simulink library "outp"  (R2021b)
settings: Solver=VariableStepAuto  StartTime=0.0  StopTime=10.0  RelTol=1e-3
undefined symbols (not defined in the file or in its folder): ENUM_PMMMODE_CHARGE, ENUM_PMMMODE_IDLE, ENUM_PMMMODE_INITIALIZE, ENUM_PMMMODE_POWERDOWN, ENUM_PMMMODE_SLEEP, Left, outp, slcm, TRUE
libraries: FVT_lib x645, hcu_lib x4, simulink x1
(part 2 of 7)

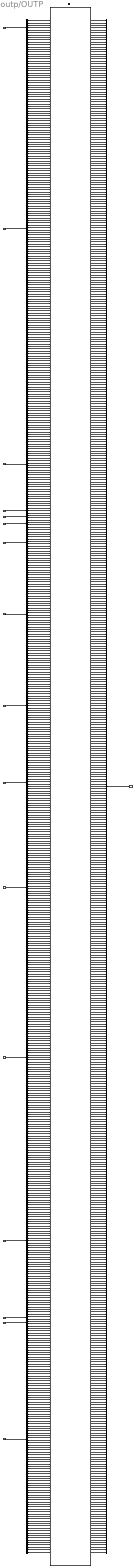
== system outp/OUTP ==
  BACC_outputs : Inport  OutDataTypeStr=Bus: BACC_outputs
  BAPM_outputs : Inport  Port=2  OutDataTypeStr=Bus: BAPM_outputs
  BBCM_outputs : Inport  Port=3  OutDataTypeStr=Bus: BBCM_outputs
  BDHP_outputs : Inport  Port=4  OutDataTypeStr=Bus: BDHP_outputs
  BDKC_outputs : Inport  Port=5  OutDataTypeStr=Bus: BDKC_outputs
  BDSC_outputs : Inport  Port=6  OutDataTypeStr=Bus: BDSC_outputs
  BNMM_outputs : Inport  Port=7  OutDataTypeStr=Bus: BNMM_outputs
  BPMM_outputs : Inport  Port=8  OutDataTypeStr=Bus: BPMM_outputs
  BSCP_outputs : Inport  Port=9  OutDataTypeStr=Bus: BSCP_outputs
  BSYS_outputs : Inport  Port=10  OutDataTypeStr=Bus: BSYS_outputs
  BTHC_outputs : Inport  Port=11  OutDataTypeStr=Bus: BTHC_outputs
  BTPM_outputs : Inport  Port=12  OutDataTypeStr=Bus: BTPM_outputs
  BTQD_outputs : Inport  Port=13  OutDataTypeStr=Bus: BTQD_outputs
  BTQR_outputs : Inport  Port=14  OutDataTypeStr=Bus: BTQR_outputs
  BV2L_outputs : Inport  Port=15  OutDataTypeStr=Bus: BV2L_outputs
  BVMC_outputs : Inport  Port=16  OutDataTypeStr=Bus: BVMC_outputs
  trig_OUTP : TriggerPort  TriggerType=function-call  VariantControl=(inherit)
  bus_creator : BusCreator  Inputs=645
  bus_selector1 : BusSelector  OutputSignals=VACC_HVTHCMSysAvail_enum,VACC_LVBattVoltSta_enum,VACC_VehHVPwrAvail4THCM_W,VACC_EHPSEnDem_enum,VACC_CACPresWarnSta_flg,VACC_CACTempWarnSta_flg,VACC_EACEnDem_enum
  bus_selector10 : BusSelector  OutputSignals=VSYS_HWVer1_cnt,VSYS_HWVer2_cnt,VSYS_HWVer3_cnt,VSYS_CarModel1_cnt,VSYS_CarModel2_cnt,VSYS_CarModel3_cnt,VSYS_ECU1_cnt,VSYS_ECU2_cnt,VSYS_Major1_cnt,VSYS_Major2_cnt,VSYS_Minor1_cnt,VSYS_Minor2_cnt,VSYS_Patch1_cnt,VSYS_Patch2_cnt,VSYS_Country1_cnt,VSYS_Country2_cnt,VSYS_Variation_cnt,VSYS_Dash1_cnt,VSYS_Change1_cnt,VSYS_Change2_cnt,VSYS_Dash2_cnt,VSYS_SHA1_cnt,VSYS_SHA2_cnt,VSYS_SHA3_cnt,VSYS_SHA4_cnt,VSYS_SHA5_cnt,VSYS_SHA6_cnt,VSYS_SHA7_cnt,VSYS_SHA8_cnt,VSYS_NvWriteReqRisingEdge_flg,VSYS_FdcSlpReqRisingEdge_flg,VSYS_FdcSlpTime_sec,VSYS_PmicBootReason_enum,VSYS_WisrBootReason_raw32,VSYS_AcoreRebootCmdACK_flg,VSYS_CurrentNmState_enum
  bus_selector11 : BusSelector  OutputSignals=VTHC_FDCompCmd_rpm,VTHC_FDSOV1Cmd_flg,VTHC_FDSOV2Cmd_flg,VTHC_FDSOV3Cmd_flg,VTHC_FDEXV1Cmd_step,VTHC_FDEXV2Cmd_step,VTHC_FDSOTXVCmd_flg,VTHC_FDFWVCmd_flg,VTHC_FDTWVCmd_pct,VTHC_FDFrWPTCHeatPwrCmd_W,VTHC_CoolgFanActDuty_pct,VTHC_FDAGSCmd_enum,VTHC_FDEWP1Cmd_enum,VTHC_FDEWP2Cmd_enum,VTHC_FDEWP3Cmd_enum,VTHC_FDFrLeAPTCHeatPwrCmd_W,VTHC_FDFrRiAPTCHeatPwrCmd_W,VTHC_FDRrAPTCHeatPwrCmd_W,VTHC_FDBlowerCmd_pct,VTHC_BatteryMode_enum,VTHC_EDriveMode_enum,VTHC_CabinMode_enum,VTHC_CCUACLampSts_flg,VTHC_CCUAutoLampSts_flg,VTHC_CCUACMaxLampSts_flg,VTHC_CCUSyncLampSts_flg,VTHC_sigAirIntenZon1St_enum,VTHC_sigWindDirZon1St_enum,VTHC_sigRecircSt_flg,VTHC_sigSetTempZon1St_C,VTHC_sigSetTempZon2St_C,VTHC_sigClntTHvBattOut_C,VTHC_sigCbnSolarLeft_W,VTHC_sigClntTHvBattIn_C,VTHC_sigCbnSolarRight_W,VTHC_sigAmbAirT_C,VTHC_sigCbnAirT_C,VTHC_ACSubMode_enum,VTHC_FDRecyAutoCmd_enum,VTHC_ACModeMem_enum,VTHC_Face_flg,VTHC_Foot_flg,VTHC_Frost_flg,VTHC_FaceM_flg,VTHC_FootM_flg,VTHC_CCUSyncSts_flg,VTHC_ACForceOFF_flg,VTHC_RecAutoFlg_flg,VTHC_AirIntenZone1M_enum,VTHC_fdefog_flg,VTHC_sigSetTempZon2StM_C,VTHC_FDCTHCMAPTCWarningSta_flg
  bus_selector12 : BusSelector  OutputSignals=VTPM_LFBatWarn_flg,VTPM_RFBatWarn_flg,VTPM_LRBatWarn_flg,VTPM_RRBatWarn_flg,VTPM_LFWheelPress_raw8,VTPM_RFWheelPress_raw8,VTPM_LRWheelPress_raw8,VTPM_RRWheelPress_raw8,VTPM_LFWheelTemp_C,VTPM_RFWheelTemp_C,VTPM_LRWheelTemp_C,VTPM_RRWheelTemp_C,VTPM_LFSensorFail_flg,VTPM_RFSensorFail_flg,VTPM_LRSensorFail_flg,VTPM_RRSensorFail_flg,VTPM_LFWheelDebug_flg,VTPM_LRWheelDebug_flg,VTPM_RFWheelDebug_flg,VTPM_RRWheelDebug_flg,VTPM_TPMSResButtAllow_flg,VTPM_TPMSCaliButtAllow_flg,VTPM_LFPressIndi_enum,VTPM_RFPressIndi_enum,VTPM_LRPressIndi_enum,VTPM_RRPressIndi_enum,VTPM_TPMSWarnIndi_enum,VTPM_LFWheelTmpIndi_flg,VTPM_RFWheelTmpIndi_flg,VTPM_LRWheelTmpIndi_flg,VTPM_RRWheelTmpIndi_flg,VTPM_LFWheelPSW_raw8,VTPM_LRWheelPSW_raw8,VTPM_RFWheelPSW_raw8,VTPM_RRWheelPSW_raw8,VTPM_CWheelTips_enum,VTPM_AutoLTips_enum,VTPM_LFSensorMode_flg,VTPM_RFSensorMode_flg,VTPM_LRSensorMode_flg,VTPM_RRSensorMode_flg,VTPM_S1ID_raw32,VTPM_S2ID_raw32,VTPM_S3ID_raw32,VTPM_S4ID_raw32,VTPM_S1L_enum,VTPM_S2L_enum,VTPM_S3L_enum,VTPM_S4L_enum,VTPM_ALFin_flg,VTPM_LFP20_raw8,VTPM_RFP20_raw8,VTPM_LRP20_raw8,VTPM_RRP20_raw8,VTPM_FAT_flg,VTPM_IDin_raw32,VTPM_S1WheelDebugALTU_pct,VTPM_S2WheelDebugALTU_pct,VTPM_S3WheelDebugALTU_pct,VTPM_S4WheelDebugALTU_pct,VTPM_ID1messageALTU_raw8,VTPM_ID2messageALTU_raw8,VTPM_ID3messageALTU_raw8,VTPM_ID4messageALTU_raw8,VTPM_Chkfin_flg,VTPM_SetIDLoc_flg,VTPM_TPMSStorge_flg,VTPM_ChkStorge_flg,VTPM_TPMSResButt_flg,VTPM_LFPindi_enum,VTPM_RFPind_enum,VTPM_LRPindi_enum,VTPM_RRPindi_enum,VTPM_WriteChkLFID_raw,VTPM_WriteChkRFID_raw,VTPM_WriteChkLRID_raw,VTPM_WriteChkRRID_raw,VTPM_WriteChkfinLFID_raw,VTPM_WriteChkfinRFID_raw,VTPM_WriteChkfinLRID_raw,VTPM_WriteChkfinRRID_raw,VTPM_Flashchkdatavalid_enum,VTPM_Flashdatavalid_enum,VTPM_unlearnSfali_flg,VTPM_unlearnSfailvalid_enum,VTPM_Prepresstempvalid_enum,VTPM_FlashS1ID_raw,VTPM_FlashS2ID_raw,VTPM_FlashS3ID_raw,VTPM_FlashS4ID_raw,VTPM_FlashIDvalid_enum
  bus_selector13 : BusSelector  OutputSignals=VTQD_ParkRequest_flg,VTQD_TqSourceFr_enum,VTQD_TqSourceRr_enum,VTQD_FrEDUAvailBrkRgnTq_Nm,VTQD_RrEDUAvailBrkRgnTq_Nm,VTQD_EVDriveMode_enum,VTQD_ShiftGearPosn_enum,VTQD_PButtonSta_enum,VTQD_FrActvDmpDisabReq_flg,VTQD_RrActvDmpDisabReq_flg,VTQD_FrRgnDecrSta_flg,VTQD_RrRgnDecrSta_flg,VTQD_DriverWhlTqDemFr_Nm,VTQD_DriverWhlTqDemRr_Nm,VTQD_FrEDUActTq_Nm,VTQD_RrEDUActTq_Nm,VTQD_FrEDURolRgnTq_Nm,VTQD_RrEDURolRgnTq_Nm,VTQD_FrEDUSpd_rpm,VTQD_RrEDUSpd_rpm,VTQD_FrEDUSpdValid_flg,VTQD_FrEDUAvailBrkRgnTqV_flg,VTQD_RrEDUSpdValid_flg,VTQD_RrEDUAvailBrkRgnTqV_flg,VTQD_RgnAbnorSta_flg,VTQD_PTCSPermSta_flg,VTQD_FrRgnPermSta_flg,VTQD_RrRgnPermSta_flg,VTQD_FrIdcMin_A,VTQD_FrIdcMax_A,VTQD_FrUdcMin_V,VTQD_FrUdcMax_V,VTQD_RrIdcMin_A,VTQD_RrIdcMax_A,VTQD_RrUdcMin_V,VTQD_RrUdcMax_V,VTQD_ReBrakeLPReq_flg,VTQD_CreepON_flg,VTQD_ActEMpTrq_pct,VTQD_ActMaxAvaEMRecpTrq_pct,VTQD_ActDriveDirect_enum,VTQD_DLEngaged_enum,VTQD_EMTrqModeDrvBrk_enum,VTQD_ActEMpTrqHrls_pct,VTQD_ActEMOutSftSpd_rpm,VTQD_DrvDemEMRtapTrq_pct,VTQD_SACtrlDev_enum,VTQD_RetSelNonEng_pct,VTQD_ShiftPgs_enum,VTQD_AccPedal1LowSW_enum,VTQD_AccPedalPos1_pct,VTQD_ParkBrakeSW_enum,VTQD_VCUVehSpd_kph,VTQD_BrakeSW_enum,VTQD_NFricPercTorq_pct,VTQD_EMParasLoss_pct,VTQD_EEC2MSGCnt_raw,VTQD_EEC2MSGCS_raw,VTQD_FDCCHAEBSRd4BRSta_enum,VTQD_FDCCHAEBSHBSwSta_enum,VTQD_FDCCHAEBSHHSwSta_enum,VTQD_FDCVCUTUpAStaSta_enum,VTQD_FDCVCUDACStatusSta_enum
  bus_selector14 : BusSelector  OutputSignals=VTQR_FrTMTqReq_Nm,VTQR_RrTMTqReq_Nm
  bus_selector15 : BusSelector  OutputSignals=VV2L_ReqOBCV2LEna_enum,VV2L_ReqV2LIVIPopup_enum
  bus_selector16 : BusSelector  OutputSignals=VVMC_FeatSetSpdFinal_raw32,VVMC_VehicleSpeed_mph,VVMC_VehicleSpeed_kph,VVMC_MeterIndSpeed_raw32,VVMC_VMCAEBCtrlAvail_flg,VVMC_VMCACCCtrlAvail_flg,VVMC_VMCCCCtrlAvail_flg,VVMC_VMCMSACtrlAvail_flg,VVMC_FeatArbitrSta_enum,VVMC_FeatReqSpd_kph,VVMC_JerkPCT_pct,VVMC_LimitPCT_pct,VVMC_FrontRearSlipRatioCtrl_flg,VVMC_RearWhlSlipRatioCtrl_flg,VVMC_SingleWhlSlipRatioCtrl_flg,VVMC_LatAccCtrl_flg,VVMC_SafetyCtrl_flg,VVMC_SPD2ACCAct_flg,VVMC_AccCalcuPID_mps2,VVMC_ISOAccLimit_mps2,VVMC_ISODecLimit_mps2,VVMC_ISOJerkLimit_mps3,VVMC_ACCRequiredAccel_mps2,VVMC_DISCReqAcc_mps2,VVMC_FeatArbitrFinal_enum,VVMC_LateralCtrl_flg,VVMC_ADASLKASta_enum,VVMC_LKAStrToqReq_Nm,VVMC_LKATOIFault_flg,VVMC_LKATOIAct_enum,VVMC_ADASAEBReq_enum,VVMC_ADASFaultSta_flg,VVMC_AEBVehHoldReq_flg,VVMC_ACCVehHoldReq_flg,VVMC_ADASDBSReq_enum,VVMC_ADASACCSta_enum,VVMC_ACCObjDist_m,VVMC_ACCObjRelSpd_mps,VVMC_TimeGapLevel_enum,VVMC_ACCJerkUpperLimit_mps3,VVMC_ACCComfortBandUpper_mps2,VVMC_ACCJerkLowerLimit_mps3,VVMC_ACCComfortBandLower_mps2,VVMC_ADASVehSpdLim_raw32,VVMC_ADASShftPosnReqA_flg,VVMC_ADASShftPosnReq_enum,VVMC_ADASForceIdle_flg,VVMC_HazardWarningReq_flg,VVMC_RightTurnLightReq_flg,VVMC_LeftTurnLightReq_flg,VVMC_ADASFCWSta_enum,VVMC_ADASLDWSta_enum,VVMC_ADASFltWrnReq_flg,VVMC_ACCObjDstLvl_enum,VVMC_ForceLowBeam_enum,VVMC_ACCTakeoverReq_flg,VVMC_ADASWarningMsg_enum,VVMC_ADASCAMSpdLim_enum,VVMC_TargetType_enum,VVMC_ADASSLIFSpdLim_enum,VVMC_LKAHODDisplayWarning_flg,VVMC_LKAHODSoundWarning_flg,VVMC_ADASLFCSta_enum,VVMC_ADASLaneModeL_enum,VVMC_ADASLaneModeR_enum,VVMC_ADASSLIFSta_enum,VVMC_ADASISASta_enum,VVMC_ADASLDWMute_flg,VVMC_ADASFCWMute_flg,VVMC_ADASLFCHandsOffWarning_enum,VVMC_LVDADisabled_flg,VVMC_LVDAMuteSta_enum,VVMC_LVDAFailinfo_flg,VVMC_LVDAWarning_flg,VVMC_LVDAACCStatusInformation_flg,VVMC_ADASLFCWarnSound_enum,VVMC_FCMACCmode_enum,VVMC_ADASLanetypeR_enum,VVMC_ADASLanetypeL_enum,VVMC_ADASLanecurveL_raw32,VVMC_ADASLanecurveR_raw32,VVMC_ADASAEBSta_enum,VVMC_FCMLDWRequest_enum,VVMC_FCMLDWFault_flg,VVMC_ACCCtrlAvail_flg,VVMC_ACCPedalOvrd_flg,VVMC_TimeGapCalcu_s,VVMC_CCCtrlSta_enum,VVMC_MSACtrlSta_enum,VVMC_APSCtrlAvail_flg,VVMC_APSStaSys_enum,VVMC_APSDecReqA_flg,VVMC_APSDecReq_mps2,VVMC_APSReq_enum,VVMC_CCMSASpdWar_flg,VVMC_IMUEnaCmd_flg
  bus_selector2 : BusSelector  OutputSignals=VAPM_VehSpeedToAPM_kph,VAPM_VehSpeedTimeOut_flg,VAPM_FSOffSw_enum,VAPM_FSOffSwTimeOut_flg,VAPM_ChrgPlugSta_enum,VAPM_PASDRMR_cm,VAPM_PASDRML_cm,VAPM_PASDRCR_cm,VAPM_PASDRCL_cm,VAPM_PASDFMR_cm,VAPM_PASDFML_cm,VAPM_PASDFCR_cm,VAPM_PASDFCL_cm,VAPM_APSDRLR_cm,VAPM_APSDRLL_cm,VAPM_APSDFLR_cm,VAPM_APSDFLL_cm,VAPM_PASAFCL_enum,VAPM_PASARMR_enum,VAPM_PASARML_enum,VAPM_PASARCR_enum,VAPM_PASARCL_enum,VAPM_PASAFMR_enum,VAPM_PASAFML_enum,VAPM_PASAFCR_enum,VAPM_USSStaRMR_flg,VAPM_USSStaRML_flg,VAPM_USSStaRLR_flg,VAPM_USSStaRLL_flg,VAPM_USSStaRCR_flg,VAPM_USSStaRCL_flg,VAPM_USSStaFMR_flg,VAPM_USSStaFML_flg,VAPM_USSStaFLR_flg,VAPM_USSStaFLL_flg,VAPM_USSStaFCR_flg,VAPM_USSStaFCL_flg,VAPM_Chime_enum,VAPM_SNSRLayout_enum,VAPM_StaFSya_flg,VAPM_ModOperation_enum,VAPM_BrkPedalPosToAPM_pct,VAPM_BrkPedalPosTimeOut_flg,VAPM_LFRawWhlSpeed_kph,VAPM_LFRawWhlSpeedTimeOut_flg,VAPM_RFRawWhlSpeed_kph,VAPM_RFRawWhlSpeedTimeOut_flg,VAPM_LRRawWhlSpeed_kph,VAPM_LRRawWhlSpeedTimeOut_flg,VAPM_RRRawWhlSpeed_kph,VAPM_RRRawWhlSpeedTimeOut_flg,VAPM_LFRawWhlSpeedV_flg,VAPM_LFRawWhlSpeedVTimeOut_flg,VAPM_RFRawWhlSpeedV_flg,VAPM_RFRawWhlSpeedVTimeOut_flg,VAPM_LRRawWhlSpeedV_flg,VAPM_LRRawWhlSpeedVTimeOut_flg,VAPM_RRRawWhlSpeedV_flg,VAPM_RRRawWhlSpeedVTimeOut_flg,VAPM_LFWhlRotDir_enum,VAPM_LFWhlRotDirTimeOut_flg,VAPM_RFWhlRotDir_enum,VAPM_RFWhlRotDirTimeOut_flg,VAPM_LRWhlRotDir_enum,VAPM_LRWhlRotDirTimeOut_flg,VAPM_RRWhlRotDir_enum,VAPM_RRWhlRotDirTimeOut_flg,VAPM_LFPulseCountV_flg,VAPM_LFPulseCountVTimeOut_flg,VAPM_RFPulseCountV_flg,VAPM_RFPulseCountVTimeOut_flg,VAPM_LRPulseCountV_flg,VAPM_LRPulseCountVTimeOut_flg,VAPM_RRPulseCountV_flg,VAPM_RRPulseCountVTimeOut_flg,VAPM_LFPulseCount_enum,VAPM_LFPulseCountTimeOut_flg,VAPM_RFPulseCount_enum,VAPM_RFPulseCountTimeOut_flg,VAPM_LRPulseCount_enum,VAPM_LRPulseCountTimeOut_flg,VAPM_RRPulseCount_enum,VAPM_RRPulseCountTimeOut_flg,VAPM_ShifterHandleCmd_enum,VAPM_ShifterHandleCmdTimeOut_flg,VAPM_DriIntend_enum,VAPM_DriIntendTimeOut_flg,VAPM_EPSAOIControl_enum,VAPM_EPSAOIControlTimeOut_flg,VAPM_SASAngle_Deg,VAPM_SASAngleTimeOut_flg,VAPM_SASSpeed_degps,VAPM_SASSpeedTimeOut_flg,VAPM_SASSpeedValid_flg,VAPM_SASSpeedValidTimeOut_flg,VAPM_SASCAL_flg,VAPM_SASCALTimeOut_flg,VAPM_SASV_flg,VAPM_SASVTimeOut_flg,VAPM_GRADE_Deg,VAPM_GRADETimeOut_flg,VAPM_YawRate_degps,VAPM_YawRateTimeOut_flg,VAPM_LatAccel_Gps,VAPM_LatAccelTimeOut_flg,VAPM_LongAccel_Gps,VAPM_LongAccelTimeOut_flg,VAPM_MCPressure_bar,VAPM_MCPressureTimeOut_flg,VAPM_YawRateV_flg,VAPM_YawRateVTimeOut_flg,VAPM_LatAccelV_flg,VAPM_LatAccelVTimeOut_flg,VAPM_LongAccelV_flg,VAPM_LongAccelVTimeOut_flg,VAPM_MCPressureV_bar,VAPM_MCPressureVTimeOut_flg,VAPM_BrkSwSta_flg,VAPM_BrkSwStaTimeOut_flg,VAPM_BrkSwV_flg,VAPM_BrkSwVTimeOut_flg,VAPM_ESCStandstill_flg,VAPM_ESCStandstillTimeOut_flg,VAPM_ESCAPSSta_enum,VAPM_ESCAPSStaTimeOut_flg,VAPM_EPBExtReleaseAvail_flg,VAPM_EPBExtReleaseAvailTimeOut_flg,VAPM_EPBExtApplyAvail_flg,VAPM_EPBExtApplyAvailTimeOut_flg,VAPM_EPBErrSta_enum,VAPM_EPBErrStaTimeOut_flg,VAPM_EPBSta_enum,VAPM_EPBStaTimeOut_flg,VAPM_AVMparkingcancel_enum,VAPM_AVMparkingcancelTimeOut_flg,VAPM_AVMparkingexcute_enum,VAPM_AVMparkingexcuteTimeOut_flg,VAPM_AVMParkingmode_enum,VAPM_AVMParkingmodeTimeOut_flg,VAPM_AVMErrSTA_flg,VAPM_AVMErrSTATimeOut_flg,VAPM_IVIStatus_flg,VAPM_IVIStatusTimeOut_flg,VAPM_CAASSw_enum,VAPM_CAASSwTimeOut_flg,VAPM_IVIScreen_enum,VAPM_IVIScreenTimeOut_flg,VAPM_ABSActiveToAPM_flg,VAPM_ABSActiveTimeOut_flg,VAPM_TCSActiveToAPM_flg,VAPM_TCSActiveTimeOut_flg,VAPM_DriverSeatBeltCmd_flg,VAPM_DriverSeatBeltCmdTimeOut_flg,VAPM_APSProgressPCT_pct,VAPM_APSRQDisplay_enum,VAPM_APSSWVer_enum,VAPM_APSHWVer_enum,VAPM_APSExitCondition_enum,VAPM_APSAngleTarget_Deg,VAPM_APSVRqEPASCtrl_flg,VAPM_APSRqEPASCtrl_flg,VAPM_CAASSta_enum
  bus_selector3 : BusSelector  OutputSignals=VBCM_HornCtrl_flg,VBCM_FRHaltBrakeSta_enum,VBCM_FRDisIntEmCmd_flg,VBCM_FROpenClosePBCmd_enum,VBCM_DoorStaSta_enum,VBCM_BrakeLamp_flg,VBCM_LDRL_flg,VBCM_RDRL_flg,VBCM_ReverseLamp_flg,VBCM_RrFogLamp_flg,VBCM_HBeam_flg,VBCM_LBeam_flg,VBCM_PosLamp_flg,VBCM_HazardSW_flg,VBCM_LTurnLP_flg,VBCM_RTurnLP_flg,VBCM_LSMLPCmd_flg,VBCM_RSMLPCmd_flg,VBCM_TurnLpLActiveCmd_flg,VBCM_TurnLpRActiveCmd_flg,VBCM_BBuzzerCmd_flg,VBCM_FrWiperL_flg,VBCM_FrWiperH_flg,VBCM_WasherCtrl_enum,VBCM_RrRmLampBrightCmd_enum,VBCM_WelcomeDemoSta_flg,VBCM_FrAtmoLampCmd_flg,VBCM_RrAtmoLampCmd_flg,VBCM_TgateHDSWLSta_flg,VBCM_TgateHDSWRSta_flg,VBCM_TgateSWLSta_flg,VBCM_TgateSWRSta_flg,VBCM_LTgateRelCmd_flg,VBCM_RTgateRelCmd_flg,VBCM_FDDoorOpen_enum,VBCM_FDDoorstate_enum
  bus_selector4 : BusSelector  OutputSignals=VDHP_ActAPSPosn_pct,VDHP_EAPS1MIN_pct,VDHP_EAPS2MIN_pct
  bus_selector5 : BusSelector  OutputSignals=VDKC_DKCTimeSN_cnt,VDKC_DKCAuthSta_enum
  bus_selector6 : BusSelector  OutputSignals=VDSC_DISCTurn_flg,VDSC_DISCTargetSpd_kph,VDSC_DISCSta_enum,VDSC_DISCButtSta_flg
  bus_selector7 : BusSelector  OutputSignals=VNMM_AllCANTxReq_flg,VNMM_NMmTxReq_flg,VNMM_Awake_enum,VNMM_CSB_flg,VNMM_ErrorState_enum,VNMM_NodeID_enum,VNMM_PNI_flg,VNMM_RptMsgReq_flg,VNMM_WakeUp_enum,VNMM_ActiveWU_flg,VNMM_SysNMmSta_enum,VNMM_NetworkReq_flg
  bus_selector8 : BusSelector  OutputSignals=VPMM_PowerUpState_enum,VPMM_PowerDownState_enum,VPMM_PowerUpFault_enum,VPMM_PowerDownFault_enum,VPMM_ActiveDischargeReq_flg,VPMM_DCDCEnaReq_flg,VPMM_DCDCVoltSetpoint_V,VPMM_HVBatCnctReq_flg,VPMM_HVSysReadyToCharge_enum,VPMM_PowerSta_enum,VPMM_LVPwrSta_flg,VPMM_HVPwrSta_flg,VPMM_SysPowerMode_enum,VPMM_FrMCUEnaReq_flg,VPMM_RrMCUEnaReq_flg,VPMM_DrivetrainSelect_enum,VPMM_DrSeatSta_enum,VPMM_PwrStaSelect_enum,VPMM_PwrStaConstraint_enum,VPMM_TCountSta_enum,VPMM_PwrUpReq_enum,VPMM_PwrDownReq_enum,VPMM_LowSOCWarn_enum,VPMM_ReVehThdChkSta_enum,VPMM_LVSysErrPwrOutErr_flg,VPMM_EvccAplusPwrUpReq_flg,VPMM_PwrStaONTOPopReq_flg,VPMM_IVIPwrStaONTOPopT_s,VPMM_LVChrgHoldTtimer_s,VPMM_LVBattChrgTimeCnt_s,VPMM_SilentChkAllowSleep_flg,VPMM_TimerAllowSleep_flg,VPMM_FDADC12VDetAvg_mV,VPMM_PMMAllowECUSleep_flg,VPMM_LVSilentChrgSta_enum,VPMM_LVSilentChrgReq_flg,VPMM_LVSilentChrgLv_enum,VPMM_CtrlFrPwrStbA1P_flg,VPMM_CtrlFrRC1_flg,VPMM_CtrlFrBMSCCUCIR_flg,VPMM_CtrlFrEDUINVERTER_flg,VPMM_HWResetSta_enum,VPMM_CtrlDrPwrStbA2_flg,VPMM_PwrStaTOSta_enum,VPMM_DCDCRlyDem_enum,VPMM_EACRlyDem_enum,VPMM_EHPSRlyDem_enum,VPMM_DCDCEnDem_enum
  bus_selector9 : BusSelector  OutputSignals=VSCP_Vehspeed_kph,VSCP_SCPBrkSwSta_flg,VSCP_AmberWnlmpSta_flg,VSCP_ABSWnlmpSta_flg,VSCP_HSAFailed_flg,VSCP_MeterIndVehSpeed_kph,VSCP_ABSFailed_flg,VSCP_ABSActive_flg,VSCP_HSAActive_flg,VSCP_RedWnlmpSta_flg,VSCP_BrkPedalPos_pct,VSCP_OpenStatusOfDoor1_enum,VSCP_OpenStatusOfDoor2_enum,VSCP_SeatBeltSwitch_enum,VSCP_triggerBAM_flg,VSCP_CFGEM1Ctrl_raw,VSCP_CFGEM1BAMTSize_raw,VSCP_CFGEM1BAMTNum_raw,VSCP_CFGEM1BAMRsv_raw,VSCP_CFGEM1BAMPGN_raw,VSCP_triggerDT_flg,VSCP_DTbyte0_raw,VSCP_DTbyte1_raw,VSCP_DTbyte2_raw,VSCP_DTbyte3_raw,VSCP_DTbyte4_raw,VSCP_DTbyte5_raw,VSCP_DTbyte6_raw,VSCP_DTbyte7_raw
  outpmodule : Subsystem
  BOUTP_outputs : Outport  OutDataTypeStr=Bus: BOUTP_outputs
  wires:
  outpmodule/33(VOUTP_USSStaRMR_flg) -> bus_creator/33
  outpmodule/32(VOUTP_PASAFCR_enum) -> bus_creator/32
  outpmodule/30(VOUTP_PASAFMR_enum) -> bus_creator/30
  outpmodule/31(VOUTP_PASAFML_enum) -> bus_creator/31
  outpmodule/29(VOUTP_PASARCL_enum) -> bus_creator/29
  outpmodule/28(VOUTP_PASARCR_enum) -> bus_creator/28
  outpmodule/25(VOUTP_PASAFCL_enum) -> bus_creator/25
  outpmodule/23(VOUTP_APSDFLR_cm) -> bus_creator/23
  outpmodule/22(VOUTP_APSDRLL_cm) -> bus_creator/22
  outpmodule/24(VOUTP_APSDFLL_cm) -> bus_creator/24
  outpmodule/21(VOUTP_APSDRLR_cm) -> bus_creator/21
  outpmodule/18(VOUTP_PASDFML_cm) -> bus_creator/18
  outpmodule/16(VOUTP_PASDRCL_cm) -> bus_creator/16
  outpmodule/13(VOUTP_PASDRMR_cm) -> bus_creator/13
  outpmodule/10(VOUTP_FSOffSw_enum) -> bus_creator/10
  outpmodule/9(VOUTP_VehSpeedTimeOut_flg) -> bus_creator/9
  outpmodule/7(VOUTP_EACEnDem_enum) -> bus_creator/7
  outpmodule/6(VOUTP_CACTempWarnSta_flg) -> bus_creator/6
  outpmodule/5(VOUTP_CACPresWarnSta_flg) -> bus_creator/5
  outpmodule/4(VOUTP_EHPSEnDem_enum) -> bus_creator/4
  outpmodule/3(VOUTP_VehHVPwrAvail4THCM_W) -> bus_creator/3
  outpmodule/1(VOUTP_HVTHCMSysAvail_enum) -> bus_creator/1
  outpmodule/378(VOUTP_FDRecyAutoCmd_enum) -> bus_creator/378
  outpmodule/377(VOUTP_ACSubMode_enum) -> bus_creator/377
  outpmodule/374(VOUTP_sigCbnSolarRight_W) -> bus_creator/374
  outpmodule/376(VOUTP_sigCbnAirT_C) -> bus_creator/376
  outpmodule/372(VOUTP_sigCbnSolarLeft_W) -> bus_creator/372
  outpmodule/371(VOUTP_sigClntTHvBattOut_C) -> bus_creator/371
  outpmodule/369(VOUTP_sigSetTempZon1St_C) -> bus_creator/369
  outpmodule/368(VOUTP_sigRecircSt_flg) -> bus_creator/368
  outpmodule/367(VOUTP_sigWindDirZon1St_enum) -> bus_creator/367
  outpmodule/365(VOUTP_CCUSyncLampSts_flg) -> bus_creator/365
  outpmodule/364(VOUTP_CCUACMaxLampSts_flg) -> bus_creator/364
  outpmodule/361(VOUTP_CabinMode_enum) -> bus_creator/361
  outpmodule/359(VOUTP_BatteryMode_enum) -> bus_creator/359
  outpmodule/360(VOUTP_EDriveMode_enum) -> bus_creator/360
  outpmodule/357(VOUTP_FDRrAPTCHeatPwrCmd_W) -> bus_creator/357
  outpmodule/354(VOUTP_FDEWP3Cmd_enum) -> bus_creator/354
  outpmodule/355(VOUTP_FDFrLeAPTCHeatPwrCmd_W) -> bus_creator/355
  outpmodule/353(VOUTP_FDEWP2Cmd_enum) -> bus_creator/353
  outpmodule/350(VOUTP_CoolgFanActDuty_pct) -> bus_creator/350
  outpmodule/347(VOUTP_FDFWVCmd_flg) -> bus_creator/347
  outpmodule/346(VOUTP_FDSOTXVCmd_flg) -> bus_creator/346
  outpmodule/345(VOUTP_FDEXV2Cmd_step) -> bus_creator/345
  outpmodule/344(VOUTP_FDEXV1Cmd_step) -> bus_creator/344
  outpmodule/343(VOUTP_FDSOV3Cmd_flg) -> bus_creator/343
  outpmodule/600(VOUTP_ADASFCWSta_enum) -> bus_creator/600
  outpmodule/381(VOUTP_Foot_flg) -> bus_creator/381
  bus_selector2/43 -> outpmodule/50(VAPM_BrkPedalPosTimeOut_flg)  "<VAPM_BrkPedalPosTimeOut_flg>"
  bus_selector2/46 -> outpmodule/53(VAPM_RFRawWhlSpeed_kph)  "<VAPM_RFRawWhlSpeed_kph>"
  bus_selector2/41 -> outpmodule/48(VAPM_ModOperation_enum)  "<VAPM_ModOperation_enum>"
  bus_selector2/40 -> outpmodule/47(VAPM_StaFSya_flg)  "<VAPM_StaFSya_flg>"
  bus_selector2/136 -> outpmodule/143(VAPM_AVMparkingexcute_enum)  "<VAPM_AVMparkingexcute_enum>"
  bus_selector2/49 -> outpmodule/56(VAPM_LRRawWhlSpeedTimeOut_flg)  "<VAPM_LRRawWhlSpeedTimeOut_flg>"
  bus_selector2/103 -> outpmodule/110(VAPM_YawRateTimeOut_flg)  "<VAPM_YawRateTimeOut_flg>"
  bus_selector2/47 -> outpmodule/54(VAPM_RFRawWhlSpeedTimeOut_flg)  "<VAPM_RFRawWhlSpeedTimeOut_flg>"
  outpmodule/373(VOUTP_sigClntTHvBattIn_C) -> bus_creator/373
  outpmodule/34(VOUTP_USSStaRML_flg) -> bus_creator/34
  bus_selector2/48 -> outpmodule/55(VAPM_LRRawWhlSpeed_kph)  "<VAPM_LRRawWhlSpeed_kph>"
  bus_selector2/45 -> outpmodule/52(VAPM_LFRawWhlSpeedTimeOut_flg)  "<VAPM_LFRawWhlSpeedTimeOut_flg>"
  outpmodule/184(VOUTP_LTurnLP_flg) -> bus_creator/184
  outpmodule/185(VOUTP_RTurnLP_flg) -> bus_creator/185
  outpmodule/183(VOUTP_HazardSW_flg) -> bus_creator/183
  outpmodule/182(VOUTP_PosLamp_flg) -> bus_creator/182
  outpmodule/178(VOUTP_ReverseLamp_flg) -> bus_creator/178
  bus_selector2/35 -> outpmodule/42(VAPM_USSStaFLL_flg)  "<VAPM_USSStaFLL_flg>"
  outpmodule/176(VOUTP_LDRL_flg) -> bus_creator/176
  outpmodule/174(VOUTP_DoorStaSta_enum) -> bus_creator/174
  outpmodule/173(VOUTP_FROpenClosePBCmd_enum) -> bus_creator/173
  outpmodule/172(VOUTP_FRDisIntEmCmd_flg) -> bus_creator/172
  outpmodule/170(VOUTP_HornCtrl_flg) -> bus_creator/170
  outpmodule/169(VOUTP_CAASSta_enum) -> bus_creator/169
  outpmodule/168(VOUTP_APSRqEPASCtrl_flg) -> bus_creator/168
  outpmodule/237(VOUTP_LVPwrSta_flg) -> bus_creator/237
  outpmodule/175(VOUTP_BrakeLamp_flg) -> bus_creator/175
  outpmodule/234(VOUTP_HVBatCnctReq_flg) -> bus_creator/234
  outpmodule/236(VOUTP_PowerSta_enum) -> bus_creator/236
  outpmodule/232(VOUTP_DCDCEnaReq_flg) -> bus_creator/232
  outpmodule/228(VOUTP_PowerDownState_enum) -> bus_creator/228
  outpmodule/225(VOUTP_SysNMmSta_enum) -> bus_creator/225
  outpmodule/224(VOUTP_ActiveWU_flg) -> bus_creator/224
  outpmodule/222(VOUTP_RptMsgReq_flg) -> bus_creator/222
  outpmodule/220(VOUTP_NodeID_enum) -> bus_creator/220
  outpmodule/218(VOUTP_CSB_flg) -> bus_creator/218
  outpmodule/217(VOUTP_Awake_enum) -> bus_creator/217
  outpmodule/216(VOUTP_NMmTxReq_flg) -> bus_creator/216
  outpmodule/215(VOUTP_AllCANTxReq_flg) -> bus_creator/215
  outpmodule/214(VOUTP_DISCButtSta_flg) -> bus_creator/214
  outpmodule/212(VOUTP_DISCTargetSpd_kph) -> bus_creator/212
  outpmodule/210(VOUTP_DKCAuthSta_enum) -> bus_creator/210
  outpmodule/207(VOUTP_EAPS1MIN_pct) -> bus_creator/207
  outpmodule/206(VOUTP_ActAPSPosn_pct) -> bus_creator/206
  outpmodule/205(VOUTP_FDDoorstate_enum) -> bus_creator/205
  outpmodule/204(VOUTP_FDDoorOpen_enum) -> bus_creator/204
  outpmodule/198(VOUTP_TgateHDSWLSta_flg) -> bus_creator/198
  outpmodule/196(VOUTP_FrAtmoLampCmd_flg) -> bus_creator/196
  outpmodule/195(VOUTP_WelcomeDemoSta_flg) -> bus_creator/195
  outpmodule/193(VOUTP_WasherCtrl_enum) -> bus_creator/193
  outpmodule/192(VOUTP_FrWiperH_flg) -> bus_creator/192
  outpmodule/190(VOUTP_BBuzzerCmd_flg) -> bus_creator/190
  outpmodule/187(VOUTP_RSMLPCmd_flg) -> bus_creator/187
  outpmodule/188(VOUTP_TurnLpLActiveCmd_flg) -> bus_creator/188
  outpmodule/272(VOUTP_EACRlyDem_enum) -> bus_creator/272
  outpmodule/270(VOUTP_PwrStaTOSta_enum) -> bus_creator/270
  outpmodule/269(VOUTP_CtrlDrPwrStbA2_flg) -> bus_creator/269
  outpmodule/267(VOUTP_CtrlFrEDUINVERTER_flg) -> bus_creator/267
  outpmodule/265(VOUTP_CtrlFrRC1_flg) -> bus_creator/265
  outpmodule/264(VOUTP_CtrlFrPwrStbA1P_flg) -> bus_creator/264
  outpmodule/262(VOUTP_LVSilentChrgReq_flg) -> bus_creator/262
  outpmodule/261(VOUTP_LVSilentChrgSta_enum) -> bus_creator/261
  outpmodule/258(VOUTP_TimerAllowSleep_flg) -> bus_creator/258
  outpmodule/259(VOUTP_FDADC12VDetAvg_mV) -> bus_creator/259
  outpmodule/257(VOUTP_SilentChkAllowSleep_flg) -> bus_creator/257
  outpmodule/256(VOUTP_LVBattChrgTimeCnt_s) -> bus_creator/256
  outpmodule/250(VOUTP_ReVehThdChkSta_enum) -> bus_creator/250
  outpmodule/249(VOUTP_LowSOCWarn_enum) -> bus_creator/249
  outpmodule/246(VOUTP_TCountSta_enum) -> bus_creator/246
  outpmodule/244(VOUTP_PwrStaSelect_enum) -> bus_creator/244
  outpmodule/245(VOUTP_PwrStaConstraint_enum) -> bus_creator/245
  outpmodule/241(VOUTP_RrMCUEnaReq_flg) -> bus_creator/241
  outpmodule/300(VOUTP_DTbyte4_raw) -> bus_creator/300
  outpmodule/294(VOUTP_CFGEM1BAMPGN_raw) -> bus_creator/294
  outpmodule/290(VOUTP_CFGEM1Ctrl_raw) -> bus_creator/290
  outpmodule/289(VOUTP_triggerBAM_flg) -> bus_creator/289
  outpmodule/288(VOUTP_SeatBeltSwitch_enum) -> bus_creator/288
  outpmodule/287(VOUTP_OpenStatusOfDoor2_enum) -> bus_creator/287
  outpmodule/285(VOUTP_BrkPedalPos_pct) -> bus_creator/285
  outpmodule/286(VOUTP_OpenStatusOfDoor1_enum) -> bus_creator/286
  outpmodule/278(VOUTP_ABSWnlmpSta_flg) -> bus_creator/278
  outpmodule/275(VOUTP_Vehspeed_kph) -> bus_creator/275
  outpmodule/274(VOUTP_DCDCEnDem_enum) -> bus_creator/274
  bus_selector10/30 -> outpmodule/333(VSYS_NvWriteReqRisingEdge_flg)  "<VSYS_NvWriteReqRisingEdge_flg>"
  bus_selector10/26 -> outpmodule/329(VSYS_SHA5_cnt)  "<VSYS_SHA5_cnt>"
  bus_selector10/25 -> outpmodule/328(VSYS_SHA4_cnt)  "<VSYS_SHA4_cnt>"
  bus_selector10/22 -> outpmodule/325(VSYS_SHA1_cnt)  "<VSYS_SHA1_cnt>"
  bus_selector10/23 -> outpmodule/326(VSYS_SHA2_cnt)  "<VSYS_SHA2_cnt>"
  bus_selector10/20 -> outpmodule/323(VSYS_Change2_cnt)  "<VSYS_Change2_cnt>"
  bus_selector10/18 -> outpmodule/321(VSYS_Dash1_cnt)  "<VSYS_Dash1_cnt>"
  bus_selector10/19 -> outpmodule/322(VSYS_Change1_cnt)  "<VSYS_Change1_cnt>"
  bus_selector10/13 -> outpmodule/316(VSYS_Patch1_cnt)  "<VSYS_Patch1_cnt>"
  outpmodule/252(VOUTP_EvccAplusPwrUpReq_flg) -> bus_creator/252
  bus_selector10/15 -> outpmodule/318(VSYS_Country1_cnt)  "<VSYS_Country1_cnt>"
  bus_selector10/16 -> outpmodule/319(VSYS_Country2_cnt)  "<VSYS_Country2_cnt>"
  bus_selector10/14 -> outpmodule/317(VSYS_Patch2_cnt)  "<VSYS_Patch2_cnt>"
  outpmodule/160(VOUTP_DriverSeatBeltCmdTimeOut_flg) -> bus_creator/160
  outpmodule/167(VOUTP_APSVRqEPASCtrl_flg) -> bus_creator/167
  outpmodule/164(VOUTP_APSHWVer_enum) -> bus_creator/164
  outpmodule/166(VOUTP_APSAngleTarget_Deg) -> bus_creator/166
  outpmodule/165(VOUTP_APSExitCondition_enum) -> bus_creator/165
  outpmodule/340(VOUTP_FDCompCmd_rpm) -> bus_creator/340
  outpmodule/337(VOUTP_WisrBootReason_raw32) -> bus_creator/337
  outpmodule/336(VOUTP_PmicBootReason_enum) -> bus_creator/336
  outpmodule/292(VOUTP_CFGEM1BAMTNum_raw) -> bus_creator/292
  outpmodule/333(VOUTP_NvWriteReqRisingEdge_flg) -> bus_creator/333
  outpmodule/331(VOUTP_SHA7_cnt) -> bus_creator/331
  outpmodule/213(VOUTP_DISCSta_enum) -> bus_creator/213
  outpmodule/332(VOUTP_SHA8_cnt) -> bus_creator/332
  outpmodule/342(VOUTP_FDSOV2Cmd_flg) -> bus_creator/342
  outpmodule/329(VOUTP_SHA5_cnt) -> bus_creator/329
  outpmodule/327(VOUTP_SHA3_cnt) -> bus_creator/327
  outpmodule/326(VOUTP_SHA2_cnt) -> bus_creator/326
  outpmodule/276(VOUTP_SCPBrkSwSta_flg) -> bus_creator/276
  outpmodule/324(VOUTP_Dash2_cnt) -> bus_creator/324
  outpmodule/323(VOUTP_Change2_cnt) -> bus_creator/323
  outpmodule/320(VOUTP_Variation_cnt) -> bus_creator/320
  outpmodule/319(VOUTP_Country2_cnt) -> bus_creator/319
  outpmodule/318(VOUTP_Country1_cnt) -> bus_creator/318
  outpmodule/313(VOUTP_Major2_cnt) -> bus_creator/313
  outpmodule/311(VOUTP_ECU2_cnt) -> bus_creator/311
  outpmodule/309(VOUTP_CarModel3_cnt) -> bus_creator/309
  outpmodule/310(VOUTP_ECU1_cnt) -> bus_creator/310
  bus_selector16/22 -> outpmodule/571(VVMC_ISOJerkLimit_mps3)  "<VVMC_ISOJerkLimit_mps3>"
  bus_selector16/21 -> outpmodule/570(VVMC_ISODecLimit_mps2)  "<VVMC_ISODecLimit_mps2>"
  bus_selector16/20 -> outpmodule/569(VVMC_ISOAccLimit_mps2)  "<VVMC_ISOAccLimit_mps2>"
  bus_selector16/90 -> outpmodule/639(VVMC_APSCtrlAvail_flg)  "<VVMC_APSCtrlAvail_flg>"
  bus_selector16/91 -> outpmodule/640(VVMC_APSStaSys_enum)  "<VVMC_APSStaSys_enum>"
  bus_selector16/92 -> outpmodule/641(VVMC_APSDecReqA_flg)  "<VVMC_APSDecReqA_flg>"
  bus_selector10/29 -> outpmodule/332(VSYS_SHA8_cnt)  "<VSYS_SHA8_cnt>"
  bus_selector16/88 -> outpmodule/637(VVMC_CCCtrlSta_enum)  "<VVMC_CCCtrlSta_enum>"
  bus_selector16/87 -> outpmodule/636(VVMC_TimeGapCalcu_s)  "<VVMC_TimeGapCalcu_s>"
  bus_selector16/84 -> outpmodule/633(VVMC_FCMLDWFault_flg)  "<VVMC_FCMLDWFault_flg>"
  bus_selector16/80 -> outpmodule/629(VVMC_ADASLanecurveL_raw32)  "<VVMC_ADASLanecurveL_raw32>"
  bus_selector16/76 -> outpmodule/625(VVMC_ADASLFCWarnSound_enum)  "<VVMC_ADASLFCWarnSound_enum>"
  bus_selector16/74 -> outpmodule/623(VVMC_LVDAWarning_flg)  "<VVMC_LVDAWarning_flg>"
  bus_selector16/71 -> outpmodule/620(VVMC_LVDADisabled_flg)  "<VVMC_LVDADisabled_flg>"
  bus_selector16/69 -> outpmodule/618(VVMC_ADASFCWMute_flg)  "<VVMC_ADASFCWMute_flg>"
  bus_selector16/65 -> outpmodule/614(VVMC_ADASLaneModeR_enum)  "<VVMC_ADASLaneModeR_enum>"
  bus_selector16/59 -> outpmodule/608(VVMC_TargetType_enum)  "<VVMC_TargetType_enum>"
  bus_selector16/56 -> outpmodule/605(VVMC_ACCTakeoverReq_flg)  "<VVMC_ACCTakeoverReq_flg>"
  bus_selector16/47 -> outpmodule/596(VVMC_ADASForceIdle_flg)  "<VVMC_ADASForceIdle_flg>"
  bus_selector16/49 -> outpmodule/598(VVMC_RightTurnLightReq_flg)  "<VVMC_RightTurnLightReq_flg>"
  bus_selector16/50 -> outpmodule/599(VVMC_LeftTurnLightReq_flg)  "<VVMC_LeftTurnLightReq_flg>"
  bus_selector16/48 -> outpmodule/597(VVMC_HazardWarningReq_flg)  "<VVMC_HazardWarningReq_flg>"
  bus_selector16/42 -> outpmodule/591(VVMC_ACCJerkLowerLimit_mps3)  "<VVMC_ACCJerkLowerLimit_mps3>"
  bus_selector16/44 -> outpmodule/593(VVMC_ADASVehSpdLim_raw32)  "<VVMC_ADASVehSpdLim_raw32>"
  bus_selector16/40 -> outpmodule/589(VVMC_ACCJerkUpperLimit_mps3)  "<VVMC_ACCJerkUpperLimit_mps3>"
  bus_selector16/37 -> outpmodule/586(VVMC_ACCObjDist_m)  "<VVMC_ACCObjDist_m>"
  bus_selector16/38 -> outpmodule/587(VVMC_ACCObjRelSpd_mps)  "<VVMC_ACCObjRelSpd_mps>"
  bus_selector16/34 -> outpmodule/583(VVMC_ACCVehHoldReq_flg)  "<VVMC_ACCVehHoldReq_flg>"
  bus_selector16/32 -> outpmodule/581(VVMC_ADASFaultSta_flg)  "<VVMC_ADASFaultSta_flg>"
  outpmodule/312(VOUTP_Major1_cnt) -> bus_creator/312
  bus_selector16/28 -> outpmodule/577(VVMC_LKAStrToqReq_Nm)  "<VVMC_LKAStrToqReq_Nm>"
  bus_selector10/21 -> outpmodule/324(VSYS_Dash2_cnt)  "<VSYS_Dash2_cnt>"
  bus_selector16/27 -> outpmodule/576(VVMC_ADASLKASta_enum)  "<VVMC_ADASLKASta_enum>"
  bus_selector16/25 -> outpmodule/574(VVMC_FeatArbitrFinal_enum)  "<VVMC_FeatArbitrFinal_enum>"
  bus_selector16/26 -> outpmodule/575(VVMC_LateralCtrl_flg)  "<VVMC_LateralCtrl_flg>"
  bus_selector2/39 -> outpmodule/46(VAPM_SNSRLayout_enum)  "<VAPM_SNSRLayout_enum>"
  outpmodule/200(VOUTP_TgateSWLSta_flg) -> bus_creator/200
  outpmodule/399(VOUTP_RRWheelPress_raw8) -> bus_creator/399
  outpmodule/394(VOUTP_LRBatWarn_flg) -> bus_creator/394
  outpmodule/392(VOUTP_LFBatWarn_flg) -> bus_creator/392
  outpmodule/391(VOUTP_FDCTHCMAPTCWarningSta_flg) -> bus_creator/391
  outpmodule/388(VOUTP_AirIntenZone1M_enum) -> bus_creator/388
  outpmodule/386(VOUTP_ACForceOFF_flg) -> bus_creator/386
  outpmodule/385(VOUTP_CCUSyncSts_flg) -> bus_creator/385
  outpmodule/384(VOUTP_FootM_flg) -> bus_creator/384
  outpmodule/383(VOUTP_FaceM_flg) -> bus_creator/383
  outpmodule/449(VOUTP_S2WheelDebugALTU_pct) -> bus_creator/449
  outpmodule/448(VOUTP_S1WheelDebugALTU_pct) -> bus_creator/448
  outpmodule/439(VOUTP_S3L_enum) -> bus_creator/439
  outpmodule/436(VOUTP_S4ID_raw32) -> bus_creator/436
  outpmodule/437(VOUTP_S1L_enum) -> bus_creator/437
  outpmodule/433(VOUTP_S1ID_raw32) -> bus_creator/433
  outpmodule/435(VOUTP_S3ID_raw32) -> bus_creator/435
  outpmodule/431(VOUTP_LRSensorMode_flg) -> bus_creator/431
  outpmodule/430(VOUTP_RFSensorMode_flg) -> bus_creator/430
  bus_selector16/52 -> outpmodule/601(VVMC_ADASLDWSta_enum)  "<VVMC_ADASLDWSta_enum>"
  outpmodule/429(VOUTP_LFSensorMode_flg) -> bus_creator/429
  outpmodule/424(VOUTP_LRWheelPSW_raw8) -> bus_creator/424
  outpmodule/419(VOUTP_LFWheelTmpIndi_flg) -> bus_creator/419
  outpmodule/420(VOUTP_RFWheelTmpIndi_flg) -> bus_creator/420
  outpmodule/418(VOUTP_TPMSWarnIndi_enum) -> bus_creator/418
  outpmodule/414(VOUTP_LFPressIndi_enum) -> bus_creator/414
  outpmodule/416(VOUTP_LRPressIndi_enum) -> bus_creator/416
  outpmodule/415(VOUTP_RFPressIndi_enum) -> bus_creator/415
  outpmodule/411(VOUTP_RRWheelDebug_flg) -> bus_creator/411
  outpmodule/412(VOUTP_TPMSResButtAllow_flg) -> bus_creator/412
  bus_selector16/86 -> outpmodule/635(VVMC_ACCPedalOvrd_flg)  "<VVMC_ACCPedalOvrd_flg>"
  outpmodule/410(VOUTP_RFWheelDebug_flg) -> bus_creator/410
  outpmodule/407(VOUTP_RRSensorFail_flg) -> bus_creator/407
  outpmodule/402(VOUTP_LRWheelTemp_C) -> bus_creator/402
  outpmodule/400(VOUTP_LFWheelTemp_C) -> bus_creator/400
  outpmodule/401(VOUTP_RFWheelTemp_C) -> bus_creator/401
  outpmodule/539(VOUTP_EEC2MSGCnt_raw) -> bus_creator/539
  outpmodule/538(VOUTP_EMParasLoss_pct) -> bus_creator/538
  outpmodule/248(VOUTP_PwrDownReq_enum) -> bus_creator/248
  outpmodule/536(VOUTP_BrakeSW_enum) -> bus_creator/536
  outpmodule/534(VOUTP_ParkBrakeSW_enum) -> bus_creator/534
  outpmodule/268(VOUTP_HWResetSta_enum) -> bus_creator/268
  outpmodule/532(VOUTP_AccPedal1LowSW_enum) -> bus_creator/532
  outpmodule/597(VOUTP_HazardWarningReq_flg) -> bus_creator/597
  bus_selector16/55 -> outpmodule/604(VVMC_ForceLowBeam_enum)  "<VVMC_ForceLowBeam_enum>"
  outpmodule/595(VOUTP_ADASShftPosnReq_enum) -> bus_creator/595
  outpmodule/592(VOUTP_ACCComfortBandLower_mps2) -> bus_creator/592
  outpmodule/593(VOUTP_ADASVehSpdLim_raw32) -> bus_creator/593
  outpmodule/591(VOUTP_ACCJerkLowerLimit_mps3) -> bus_creator/591
  outpmodule/181(VOUTP_LBeam_flg) -> bus_creator/181
  outpmodule/589(VOUTP_ACCJerkUpperLimit_mps3) -> bus_creator/589
  outpmodule/588(VOUTP_TimeGapLevel_enum) -> bus_creator/588
  outpmodule/587(VOUTP_ACCObjRelSpd_mps) -> bus_creator/587
  outpmodule/583(VOUTP_ACCVehHoldReq_flg) -> bus_creator/583
  outpmodule/298(VOUTP_DTbyte2_raw) -> bus_creator/298
  outpmodule/581(VOUTP_ADASFaultSta_flg) -> bus_creator/581
  outpmodule/576(VOUTP_ADASLKASta_enum) -> bus_creator/576
  outpmodule/570(VOUTP_ISODecLimit_mps2) -> bus_creator/570
  outpmodule/594(VOUTP_ADASShftPosnReqA_flg) -> bus_creator/594
  outpmodule/567(VOUTP_SPD2ACCAct_flg) -> bus_creator/567
  outpmodule/566(VOUTP_SafetyCtrl_flg) -> bus_creator/566
  outpmodule/563(VOUTP_RearWhlSlipRatioCtrl_flg) -> bus_creator/563
  outpmodule/558(VOUTP_FeatArbitrSta_enum) -> bus_creator/558
  outpmodule/560(VOUTP_JerkPCT_pct) -> bus_creator/560
  outpmodule/559(VOUTP_FeatReqSpd_kph) -> bus_creator/559
  outpmodule/551(VOUTP_VehicleSpeed_mph) -> bus_creator/551
  outpmodule/549(VOUTP_ReqV2LIVIPopup_enum) -> bus_creator/549
  outpmodule/548(VOUTP_ReqOBCV2LEna_enum) -> bus_creator/548
  outpmodule/643(VOUTP_APSReq_enum) -> bus_creator/643
  outpmodule/397(VOUTP_RFWheelPress_raw8) -> bus_creator/397
  outpmodule/162(VOUTP_APSRQDisplay_enum) -> bus_creator/162
  outpmodule/645(VOUTP_IMUEnaCmd_flg) -> bus_creator/645
  outpmodule/639(VOUTP_APSCtrlAvail_flg) -> bus_creator/639
  outpmodule/637(VOUTP_CCCtrlSta_enum) -> bus_creator/637
  bus_selector2/34 -> outpmodule/41(VAPM_USSStaFLR_flg)  "<VAPM_USSStaFLR_flg>"
  bus_selector2/22 -> outpmodule/29(VAPM_PASARCL_enum)  "<VAPM_PASARCL_enum>"
  bus_selector2/20 -> outpmodule/27(VAPM_PASARML_enum)  "<VAPM_PASARML_enum>"
  bus_selector2/21 -> outpmodule/28(VAPM_PASARCR_enum)  "<VAPM_PASARCR_enum>"
  bus_selector16/39 -> outpmodule/588(VVMC_TimeGapLevel_enum)  "<VVMC_TimeGapLevel_enum>"
  bus_selector2/19 -> outpmodule/26(VAPM_PASARMR_enum)  "<VAPM_PASARMR_enum>"
  bus_selector2/18 -> outpmodule/25(VAPM_PASAFCL_enum)  "<VAPM_PASAFCL_enum>"
  bus_selector2/16 -> outpmodule/23(VAPM_APSDFLR_cm)  "<VAPM_APSDFLR_cm>"
  bus_selector2/14 -> outpmodule/21(VAPM_APSDRLR_cm)  "<VAPM_APSDRLR_cm>"
  bus_selector2/13 -> outpmodule/20(VAPM_PASDFCL_cm)  "<VAPM_PASDFCL_cm>"
  BACC_outputs/1 -> bus_selector1/1
  bus_selector1/5 -> outpmodule/5(VACC_CACPresWarnSta_flg)  "<VACC_CACPresWarnSta_flg>"
  bus_selector1/3 -> outpmodule/3(VACC_VehHVPwrAvail4THCM_W)  "<VACC_VehHVPwrAvail4THCM_W>"
  bus_selector1/1 -> outpmodule/1(VACC_HVTHCMSysAvail_enum)  "<VACC_HVTHCMSysAvail_enum>"
  outpmodule/307(VOUTP_CarModel1_cnt) -> bus_creator/307
  outpmodule/306(VOUTP_HWVer3_cnt) -> bus_creator/306
  outpmodule/304(VOUTP_HWVer1_cnt) -> bus_creator/304
  bus_selector16/53 -> outpmodule/602(VVMC_ADASFltWrnReq_flg)  "<VVMC_ADASFltWrnReq_flg>"
  outpmodule/302(VOUTP_DTbyte6_raw) -> bus_creator/302
  bus_selector10/24 -> outpmodule/327(VSYS_SHA3_cnt)  "<VSYS_SHA3_cnt>"
  outpmodule/61(VOUTP_RFRawWhlSpeedV_flg) -> bus_creator/61
  outpmodule/60(VOUTP_LFRawWhlSpeedVTimeOut_flg) -> bus_creator/60
  outpmodule/565(VOUTP_LatAccCtrl_flg) -> bus_creator/565
  outpmodule/57(VOUTP_RRRawWhlSpeed_kph) -> bus_creator/57
  outpmodule/51(VOUTP_LFRawWhlSpeed_kph) -> bus_creator/51
  outpmodule/48(VOUTP_ModOperation_enum) -> bus_creator/48
  outpmodule/585(VOUTP_ADASACCSta_enum) -> bus_creator/585
  outpmodule/47(VOUTP_StaFSya_flg) -> bus_creator/47
  bus_selector2/23 -> outpmodule/30(VAPM_PASAFMR_enum)  "<VAPM_PASAFMR_enum>"
  outpmodule/46(VOUTP_SNSRLayout_enum) -> bus_creator/46
  outpmodule/44(VOUTP_USSStaFCL_flg) -> bus_creator/44
  outpmodule/42(VOUTP_USSStaFLL_flg) -> bus_creator/42
  outpmodule/578(VOUTP_LKATOIFault_flg) -> bus_creator/578
  outpmodule/39(VOUTP_USSStaFMR_flg) -> bus_creator/39
  outpmodule/36(VOUTP_USSStaRLL_flg) -> bus_creator/36
  outpmodule/35(VOUTP_USSStaRLR_flg) -> bus_creator/35
  outpmodule/110(VOUTP_YawRateTimeOut_flg) -> bus_creator/110
  bus_selector2/15 -> outpmodule/22(VAPM_APSDRLL_cm)  "<VAPM_APSDRLL_cm>"
  outpmodule/111(VOUTP_LatAccel_Gps) -> bus_creator/111
  outpmodule/109(VOUTP_YawRate_degps) -> bus_creator/109
  outpmodule/108(VOUTP_GRADETimeOut_flg) -> bus_creator/108
  bus_selector16/41 -> outpmodule/590(VVMC_ACCComfortBandUpper_mps2)  "<VVMC_ACCComfortBandUpper_mps2>"
  outpmodule/328(VOUTP_SHA4_cnt) -> bus_creator/328
  outpmodule/106(VOUTP_SASVTimeOut_flg) -> bus_creator/106
  outpmodule/574(VOUTP_FeatArbitrFinal_enum) -> bus_creator/574
  outpmodule/105(VOUTP_SASV_flg) -> bus_creator/105
  outpmodule/103(VOUTP_SASCAL_flg) -> bus_creator/103
  outpmodule/642(VOUTP_APSDecReq_mps2) -> bus_creator/642
  outpmodule/101(VOUTP_SASSpeedValid_flg) -> bus_creator/101
  outpmodule/97(VOUTP_SASAngle_Deg) -> bus_creator/97
  outpmodule/98(VOUTP_SASAngleTimeOut_flg) -> bus_creator/98
  outpmodule/584(VOUTP_ADASDBSReq_enum) -> bus_creator/584
  outpmodule/96(VOUTP_EPSAOIControlTimeOut_flg) -> bus_creator/96
  outpmodule/93(VOUTP_DriIntend_enum) -> bus_creator/93
  outpmodule/92(VOUTP_ShifterHandleCmdTimeOut_flg) -> bus_creator/92
  outpmodule/91(VOUTP_ShifterHandleCmd_enum) -> bus_creator/91
  outpmodule/579(VOUTP_LKATOIAct_enum) -> bus_creator/579
  outpmodule/88(VOUTP_LRPulseCountTimeOut_flg) -> bus_creator/88
  outpmodule/291(VOUTP_CFGEM1BAMTSize_raw) -> bus_creator/291
  bus_selector16/85 -> outpmodule/634(VVMC_ACCCtrlAvail_flg)  "<VVMC_ACCCtrlAvail_flg>"
  outpmodule/86(VOUTP_RFPulseCountTimeOut_flg) -> bus_creator/86
  bus_selector16/68 -> outpmodule/617(VVMC_ADASLDWMute_flg)  "<VVMC_ADASLDWMute_flg>"
  outpmodule/84(VOUTP_LFPulseCountTimeOut_flg) -> bus_creator/84
  bus_selector16/29 -> outpmodule/578(VVMC_LKATOIFault_flg)  "<VVMC_LKATOIFault_flg>"
  bus_selector5/1 -> outpmodule/209(VDKC_DKCTimeSN_cnt)  "<VDKC_DKCTimeSN_cnt>"
  outpmodule/82(VOUTP_RRPulseCountVTimeOut_flg) -> bus_creator/82
  outpmodule/83(VOUTP_LFPulseCount_enum) -> bus_creator/83
  outpmodule/78(VOUTP_RFPulseCountVTimeOut_flg) -> bus_creator/78
  outpmodule/77(VOUTP_RFPulseCountV_flg) -> bus_creator/77
  outpmodule/79(VOUTP_LRPulseCountV_flg) -> bus_creator/79
  outpmodule/75(VOUTP_LFPulseCountV_flg) -> bus_creator/75
  outpmodule/73(VOUTP_RRWhlRotDir_enum) -> bus_creator/73
  outpmodule/74(VOUTP_RRWhlRotDirTimeOut_flg) -> bus_creator/74
  outpmodule/65(VOUTP_RRRawWhlSpeedV_flg) -> bus_creator/65
  outpmodule/66(VOUTP_RRRawWhlSpeedVTimeOut_flg) -> bus_creator/66
  outpmodule/63(VOUTP_LRRawWhlSpeedV_flg) -> bus_creator/63
  outpmodule/64(VOUTP_LRRawWhlSpeedVTimeOut_flg) -> bus_creator/64
  outpmodule/53(VOUTP_RFRawWhlSpeed_kph) -> bus_creator/53
  outpmodule/452(VOUTP_ID1messageALTU_raw8) -> bus_creator/452
  outpmodule/526(VOUTP_ActEMpTrqHrls_pct) -> bus_creator/526
  outpmodule/586(VOUTP_ACCObjDist_m) -> bus_creator/586
  outpmodule/524(VOUTP_DLEngaged_enum) -> bus_creator/524
  outpmodule/240(VOUTP_FrMCUEnaReq_flg) -> bus_creator/240
  outpmodule/518(VOUTP_RrUdcMax_V) -> bus_creator/518
  outpmodule/520(VOUTP_CreepON_flg) -> bus_creator/520
  outpmodule/516(VOUTP_RrIdcMax_A) -> bus_creator/516
  outpmodule/510(VOUTP_RrRgnPermSta_flg) -> bus_creator/510
  outpmodule/511(VOUTP_FrIdcMin_A) -> bus_creator/511
  outpmodule/387(VOUTP_RecAutoFlg_flg) -> bus_creator/387
  outpmodule/509(VOUTP_FrRgnPermSta_flg) -> bus_creator/509
  outpmodule/504(VOUTP_FrEDUAvailBrkRgnTqV_flg) -> bus_creator/504
  outpmodule/11(VOUTP_FSOffSwTimeOut_flg) -> bus_creator/11
  outpmodule/505(VOUTP_RrEDUSpdValid_flg) -> bus_creator/505
  outpmodule/284(VOUTP_RedWnlmpSta_flg) -> bus_creator/284
  outpmodule/227(VOUTP_PowerUpState_enum) -> bus_creator/227
  outpmodule/502(VOUTP_RrEDUSpd_rpm) -> bus_creator/502
  outpmodule/501(VOUTP_FrEDUSpd_rpm) -> bus_creator/501
  outpmodule/444(VOUTP_LRP20_raw8) -> bus_creator/444
  outpmodule/62(VOUTP_RFRawWhlSpeedVTimeOut_flg) -> bus_creator/62
  bus_selector16/45 -> outpmodule/594(VVMC_ADASShftPosnReqA_flg)  "<VVMC_ADASShftPosnReqA_flg>"
  outpmodule/494(VOUTP_RrRgnDecrSta_flg) -> bus_creator/494
  outpmodule/495(VOUTP_DriverWhlTqDemFr_Nm) -> bus_creator/495
  outpmodule/490(VOUTP_PButtonSta_enum) -> bus_creator/490
  outpmodule/491(VOUTP_FrActvDmpDisabReq_flg) -> bus_creator/491
  outpmodule/487(VOUTP_RrEDUAvailBrkRgnTq_Nm) -> bus_creator/487
  outpmodule/481(VOUTP_FlashS4ID_raw) -> bus_creator/481
  outpmodule/480(VOUTP_FlashS3ID_raw) -> bus_creator/480
  outpmodule/478(VOUTP_FlashS1ID_raw) -> bus_creator/478
  outpmodule/477(VOUTP_Prepresstempvalid_enum) -> bus_creator/477
  outpmodule/479(VOUTP_FlashS2ID_raw) -> bus_creator/479
  outpmodule/476(VOUTP_unlearnSfailvalid_enum) -> bus_creator/476
  outpmodule/474(VOUTP_Flashdatavalid_enum) -> bus_creator/474
  outpmodule/408(VOUTP_LFWheelDebug_flg) -> bus_creator/408
  outpmodule/470(VOUTP_WriteChkfinRFID_raw) -> bus_creator/470
  bus_selector10/17 -> outpmodule/320(VSYS_Variation_cnt)  "<VSYS_Variation_cnt>"
  outpmodule/37(VOUTP_USSStaRCR_flg) -> bus_creator/37
  outpmodule/469(VOUTP_WriteChkfinLFID_raw) -> bus_creator/469
  bus_selector16/61 -> outpmodule/610(VVMC_LKAHODDisplayWarning_flg)  "<VVMC_LKAHODDisplayWarning_flg>"
  outpmodule/465(VOUTP_WriteChkLFID_raw) -> bus_creator/465
  outpmodule/467(VOUTP_WriteChkLRID_raw) -> bus_creator/467
  outpmodule/445(VOUTP_RRP20_raw8) -> bus_creator/445
  outpmodule/466(VOUTP_WriteChkRFID_raw) -> bus_creator/466
  outpmodule/459(VOUTP_ChkStorge_flg) -> bus_creator/459
  outpmodule/239(VOUTP_SysPowerMode_enum) -> bus_creator/239
  outpmodule/458(VOUTP_TPMSStorge_flg) -> bus_creator/458
  outpmodule/636(VOUTP_TimeGapCalcu_s) -> bus_creator/636
  outpmodule/409(VOUTP_LRWheelDebug_flg) -> bus_creator/409
  bus_selector2/25 -> outpmodule/32(VAPM_PASAFCR_enum)  "<VAPM_PASAFCR_enum>"
  bus_selector2/129 -> outpmodule/136(VAPM_EPBExtApplyAvailTimeOut_flg)  "<VAPM_EPBExtApplyAvailTimeOut_flg>"
  outpmodule/271(VOUTP_DCDCRlyDem_enum) -> bus_creator/271
  outpmodule/186(VOUTP_LSMLPCmd_flg) -> bus_creator/186
  outpmodule/550(VOUTP_FeatSetSpdFinal_raw32) -> bus_creator/550
  bus_selector2/128 -> outpmodule/135(VAPM_EPBExtApplyAvail_flg)  "<VAPM_EPBExtApplyAvail_flg>"
  outpmodule/76(VOUTP_LFPulseCountVTimeOut_flg) -> bus_creator/76
  bus_selector2/131 -> outpmodule/138(VAPM_EPBErrStaTimeOut_flg)  "<VAPM_EPBErrStaTimeOut_flg>"
  bus_selector2/126 -> outpmodule/133(VAPM_EPBExtReleaseAvail_flg)  "<VAPM_EPBExtReleaseAvail_flg>"
  outpmodule/382(VOUTP_Frost_flg) -> bus_creator/382
  bus_selector2/132 -> outpmodule/139(VAPM_EPBSta_enum)  "<VAPM_EPBSta_enum>"
  bus_selector2/125 -> outpmodule/132(VAPM_ESCAPSStaTimeOut_flg)  "<VAPM_ESCAPSStaTimeOut_flg>"
  bus_selector2/123 -> outpmodule/130(VAPM_ESCStandstillTimeOut_flg)  "<VAPM_ESCStandstillTimeOut_flg>"
  bus_selector2/124 -> outpmodule/131(VAPM_ESCAPSSta_enum)  "<VAPM_ESCAPSSta_enum>"
  outpmodule/209(VOUTP_DKCTimeSN_cnt) -> bus_creator/209
  outpmodule/562(VOUTP_FrontRearSlipRatioCtrl_flg) -> bus_creator/562
  outpmodule/280(VOUTP_MeterIndVehSpeed_kph) -> bus_creator/280
  outpmodule/471(VOUTP_WriteChkfinLRID_raw) -> bus_creator/471
  bus_selector2/118 -> outpmodule/125(VAPM_BrkSwSta_flg)  "<VAPM_BrkSwSta_flg>"
  bus_selector16/57 -> outpmodule/606(VVMC_ADASWarningMsg_enum)  "<VVMC_ADASWarningMsg_enum>"
  bus_selector2/122 -> outpmodule/129(VAPM_ESCStandstill_flg)  "<VAPM_ESCStandstill_flg>"
  outpmodule/375(VOUTP_sigAmbAirT_C) -> bus_creator/375
  bus_selector2/120 -> outpmodule/127(VAPM_BrkSwV_flg)  "<VAPM_BrkSwV_flg>"
  outpmodule/171(VOUTP_FRHaltBrakeSta_enum) -> bus_creator/171
  outpmodule/71(VOUTP_LRWhlRotDir_enum) -> bus_creator/71
  bus_selector2/116 -> outpmodule/123(VAPM_MCPressureV_bar)  "<VAPM_MCPressureV_bar>"
  bus_selector2/121 -> outpmodule/128(VAPM_BrkSwVTimeOut_flg)  "<VAPM_BrkSwVTimeOut_flg>"
  outpmodule/438(VOUTP_S2L_enum) -> bus_creator/438
  bus_selector2/115 -> outpmodule/122(VAPM_LongAccelVTimeOut_flg)  "<VAPM_LongAccelVTimeOut_flg>"
  bus_selector2/119 -> outpmodule/126(VAPM_BrkSwStaTimeOut_flg)  "<VAPM_BrkSwStaTimeOut_flg>"
  bus_selector2/111 -> outpmodule/118(VAPM_YawRateVTimeOut_flg)  "<VAPM_YawRateVTimeOut_flg>"
  outpmodule/50(VOUTP_BrkPedalPosTimeOut_flg) -> bus_creator/50
  bus_selector2/110 -> outpmodule/117(VAPM_YawRateV_flg)  "<VAPM_YawRateV_flg>"
  bus_selector2/109 -> outpmodule/116(VAPM_MCPressureTimeOut_flg)  "<VAPM_MCPressureTimeOut_flg>"
  bus_selector2/112 -> outpmodule/119(VAPM_LatAccelV_flg)  "<VAPM_LatAccelV_flg>"
  bus_selector2/106 -> outpmodule/113(VAPM_LongAccel_Gps)  "<VAPM_LongAccel_Gps>"
  outpmodule/325(VOUTP_SHA1_cnt) -> bus_creator/325
  outpmodule/486(VOUTP_FrEDUAvailBrkRgnTq_Nm) -> bus_creator/486
  bus_selector2/108 -> outpmodule/115(VAPM_MCPressure_bar)  "<VAPM_MCPressure_bar>"
  outpmodule/282(VOUTP_ABSActive_flg) -> bus_creator/282
  outpmodule/19(VOUTP_PASDFCR_cm) -> bus_creator/19
  bus_selector2/105 -> outpmodule/112(VAPM_LatAccelTimeOut_flg)  "<VAPM_LatAccelTimeOut_flg>"
  bus_selector2/104 -> outpmodule/111(VAPM_LatAccel_Gps)  "<VAPM_LatAccel_Gps>"
  outpmodule/403(VOUTP_RRWheelTemp_C) -> bus_creator/403
  outpmodule/94(VOUTP_DriIntendTimeOut_flg) -> bus_creator/94
  bus_selector2/107 -> outpmodule/114(VAPM_LongAccelTimeOut_flg)  "<VAPM_LongAccelTimeOut_flg>"
  bus_selector2/93 -> outpmodule/100(VAPM_SASSpeedTimeOut_flg)  "<VAPM_SASSpeedTimeOut_flg>"
  outpmodule/41(VOUTP_USSStaFLR_flg) -> bus_creator/41
  bus_selector2/98 -> outpmodule/105(VAPM_SASV_flg)  "<VAPM_SASV_flg>"
  outpmodule/553(VOUTP_MeterIndSpeed_raw32) -> bus_creator/553
  bus_selector2/100 -> outpmodule/107(VAPM_GRADE_Deg)  "<VAPM_GRADE_Deg>"
  outpmodule/446(VOUTP_FAT_flg) -> bus_creator/446
  outpmodule/189(VOUTP_TurnLpRActiveCmd_flg) -> bus_creator/189
  bus_selector2/99 -> outpmodule/106(VAPM_SASVTimeOut_flg)  "<VAPM_SASVTimeOut_flg>"
  bus_selector2/97 -> outpmodule/104(VAPM_SASCALTimeOut_flg)  "<VAPM_SASCALTimeOut_flg>"
  outpmodule/255(VOUTP_LVChrgHoldTtimer_s) -> bus_creator/255
  bus_selector2/96 -> outpmodule/103(VAPM_SASCAL_flg)  "<VAPM_SASCAL_flg>"
  bus_selector2/94 -> outpmodule/101(VAPM_SASSpeedValid_flg)  "<VAPM_SASSpeedValid_flg>"
  bus_selector2/88 -> outpmodule/95(VAPM_EPSAOIControl_enum)  "<VAPM_EPSAOIControl_enum>"
  bus_selector2/91 -> outpmodule/98(VAPM_SASAngleTimeOut_flg)  "<VAPM_SASAngleTimeOut_flg>"
  bus_selector2/92 -> outpmodule/99(VAPM_SASSpeed_degps)  "<VAPM_SASSpeed_degps>"
  outpmodule/163(VOUTP_APSSWVer_enum) -> bus_creator/163
  outpmodule/596(VOUTP_ADASForceIdle_flg) -> bus_creator/596
  bus_selector2/87 -> outpmodule/94(VAPM_DriIntendTimeOut_flg)  "<VAPM_DriIntendTimeOut_flg>"
  bus_selector2/90 -> outpmodule/97(VAPM_SASAngle_Deg)  "<VAPM_SASAngle_Deg>"
  outpmodule/112(VOUTP_LatAccelTimeOut_flg) -> bus_creator/112
  outpmodule/483(VOUTP_ParkRequest_flg) -> bus_creator/483
  bus_selector2/89 -> outpmodule/96(VAPM_EPSAOIControlTimeOut_flg)  "<VAPM_EPSAOIControlTimeOut_flg>"
  bus_selector2/86 -> outpmodule/93(VAPM_DriIntend_enum)  "<VAPM_DriIntend_enum>"
  bus_selector2/83 -> outpmodule/90(VAPM_RRPulseCountTimeOut_flg)  "<VAPM_RRPulseCountTimeOut_flg>"
  outpmodule/87(VOUTP_LRPulseCount_enum) -> bus_creator/87
  bus_selector2/79 -> outpmodule/86(VAPM_RFPulseCountTimeOut_flg)  "<VAPM_RFPulseCountTimeOut_flg>"
  bus_selector2/82 -> outpmodule/89(VAPM_RRPulseCount_enum)  "<VAPM_RRPulseCount_enum>"
  bus_selector2/77 -> outpmodule/84(VAPM_LFPulseCountTimeOut_flg)  "<VAPM_LFPulseCountTimeOut_flg>"
  outpmodule/533(VOUTP_AccPedalPos1_pct) -> bus_creator/533
  bus_selector2/81 -> outpmodule/88(VAPM_LRPulseCountTimeOut_flg)  "<VAPM_LRPulseCountTimeOut_flg>"
  bus_selector2/75 -> outpmodule/82(VAPM_RRPulseCountVTimeOut_flg)  "<VAPM_RRPulseCountVTimeOut_flg>"
  bus_selector2/80 -> outpmodule/87(VAPM_LRPulseCount_enum)  "<VAPM_LRPulseCount_enum>"
  bus_selector2/73 -> outpmodule/80(VAPM_LRPulseCountVTimeOut_flg)  "<VAPM_LRPulseCountVTimeOut_flg>"
  bus_selector2/74 -> outpmodule/81(VAPM_RRPulseCountV_flg)  "<VAPM_RRPulseCountV_flg>"
  outpmodule/67(VOUTP_LFWhlRotDir_enum) -> bus_creator/67
  bus_selector2/69 -> outpmodule/76(VAPM_LFPulseCountVTimeOut_flg)  "<VAPM_LFPulseCountVTimeOut_flg>"
  outpmodule/356(VOUTP_FDFrRiAPTCHeatPwrCmd_W) -> bus_creator/356
  bus_selector2/68 -> outpmodule/75(VAPM_LFPulseCountV_flg)  "<VAPM_LFPulseCountV_flg>"
  bus_selector16/51 -> outpmodule/600(VVMC_ADASFCWSta_enum)  "<VVMC_ADASFCWSta_enum>"
  bus_selector2/71 -> outpmodule/78(VAPM_RFPulseCountVTimeOut_flg)  "<VAPM_RFPulseCountVTimeOut_flg>"
  bus_selector2/70 -> outpmodule/77(VAPM_RFPulseCountV_flg)  "<VAPM_RFPulseCountV_flg>"
  bus_selector16/30 -> outpmodule/579(VVMC_LKATOIAct_enum)  "<VVMC_LKATOIAct_enum>"
  bus_selector2/65 -> outpmodule/72(VAPM_LRWhlRotDirTimeOut_flg)  "<VAPM_LRWhlRotDirTimeOut_flg>"
  bus_selector2/66 -> outpmodule/73(VAPM_RRWhlRotDir_enum)  "<VAPM_RRWhlRotDir_enum>"
  outpmodule/305(VOUTP_HWVer2_cnt) -> bus_creator/305
  bus_selector2/67 -> outpmodule/74(VAPM_RRWhlRotDirTimeOut_flg)  "<VAPM_RRWhlRotDirTimeOut_flg>"
  outpmodule/517(VOUTP_RrUdcMin_V) -> bus_creator/517
  bus_selector2/64 -> outpmodule/71(VAPM_LRWhlRotDir_enum)  "<VAPM_LRWhlRotDir_enum>"
  bus_selector2/59 -> outpmodule/66(VAPM_RRRawWhlSpeedVTimeOut_flg)  "<VAPM_RRRawWhlSpeedVTimeOut_flg>"
  bus_selector2/58 -> outpmodule/65(VAPM_RRRawWhlSpeedV_flg)  "<VAPM_RRRawWhlSpeedV_flg>"
  bus_selector2/101 -> outpmodule/108(VAPM_GRADETimeOut_flg)  "<VAPM_GRADETimeOut_flg>"
  bus_selector16/81 -> outpmodule/630(VVMC_ADASLanecurveR_raw32)  "<VVMC_ADASLanecurveR_raw32>"
  outpmodule/519(VOUTP_ReBrakeLPReq_flg) -> bus_creator/519
  bus_selector2/57 -> outpmodule/64(VAPM_LRRawWhlSpeedVTimeOut_flg)  "<VAPM_LRRawWhlSpeedVTimeOut_flg>"
  outpmodule/544(VOUTP_FDCVCUTUpAStaSta_enum) -> bus_creator/544
  outpmodule/221(VOUTP_PNI_flg) -> bus_creator/221
  bus_selector2/52 -> outpmodule/59(VAPM_LFRawWhlSpeedV_flg)  "<VAPM_LFRawWhlSpeedV_flg>"
  bus_selector16/33 -> outpmodule/582(VVMC_AEBVehHoldReq_flg)  "<VVMC_AEBVehHoldReq_flg>"
  outpmodule/314(VOUTP_Minor1_cnt) -> bus_creator/314
  bus_selector2/51 -> outpmodule/58(VAPM_RRRawWhlSpeedTimeOut_flg)  "<VAPM_RRRawWhlSpeedTimeOut_flg>"
  bus_selector16/63 -> outpmodule/612(VVMC_ADASLFCSta_enum)  "<VVMC_ADASLFCSta_enum>"
  bus_selector2/56 -> outpmodule/63(VAPM_LRRawWhlSpeedV_flg)  "<VAPM_LRRawWhlSpeedV_flg>"
  bus_selector2/53 -> outpmodule/60(VAPM_LFRawWhlSpeedVTimeOut_flg)  "<VAPM_LFRawWhlSpeedVTimeOut_flg>"
  bus_selector2/138 -> outpmodule/145(VAPM_AVMParkingmode_enum)  "<VAPM_AVMParkingmode_enum>"
  outpmodule/177(VOUTP_RDRL_flg) -> bus_creator/177
  BBCM_outputs/1 -> bus_selector3/1
  bus_selector4/2 -> outpmodule/207(VDHP_EAPS1MIN_pct)  "<VDHP_EAPS1MIN_pct>"
  bus_selector16/82 -> outpmodule/631(VVMC_ADASAEBSta_enum)  "<VVMC_ADASAEBSta_enum>"
  bus_selector3/34 -> outpmodule/203(VBCM_RTgateRelCmd_flg)  "<VBCM_RTgateRelCmd_flg>"
  outpmodule/72(VOUTP_LRWhlRotDirTimeOut_flg) -> bus_creator/72
  outpmodule/521(VOUTP_ActEMpTrq_pct) -> bus_creator/521
  bus_selector3/32 -> outpmodule/201(VBCM_TgateSWRSta_flg)  "<VBCM_TgateSWRSta_flg>"
  outpmodule/417(VOUTP_RRPressIndi_enum) -> bus_creator/417
  bus_selector3/33 -> outpmodule/202(VBCM_LTgateRelCmd_flg)  "<VBCM_LTgateRelCmd_flg>"
  bus_selector3/29 -> outpmodule/198(VBCM_TgateHDSWLSta_flg)  "<VBCM_TgateHDSWLSta_flg>"
  bus_selector16/72 -> outpmodule/621(VVMC_LVDAMuteSta_enum)  "<VVMC_LVDAMuteSta_enum>"
  bus_selector3/25 -> outpmodule/194(VBCM_RrRmLampBrightCmd_enum)  "<VBCM_RrRmLampBrightCmd_enum>"
  bus_selector3/24 -> outpmodule/193(VBCM_WasherCtrl_enum)  "<VBCM_WasherCtrl_enum>"
  outpmodule/557(VOUTP_VMCMSACtrlAvail_flg) -> bus_creator/557
  bus_selector3/23 -> outpmodule/192(VBCM_FrWiperH_flg)  "<VBCM_FrWiperH_flg>"
  bus_selector16/46 -> outpmodule/595(VVMC_ADASShftPosnReq_enum)  "<VVMC_ADASShftPosnReq_enum>"
  bus_selector3/15 -> outpmodule/184(VBCM_LTurnLP_flg)  "<VBCM_LTurnLP_flg>"
  bus_selector3/18 -> outpmodule/187(VBCM_RSMLPCmd_flg)  "<VBCM_RSMLPCmd_flg>"
  bus_selector3/11 -> outpmodule/180(VBCM_HBeam_flg)  "<VBCM_HBeam_flg>"
  bus_selector3/9 -> outpmodule/178(VBCM_ReverseLamp_flg)  "<VBCM_ReverseLamp_flg>"
  bus_selector3/8 -> outpmodule/177(VBCM_RDRL_flg)  "<VBCM_RDRL_flg>"
  outpmodule/580(VOUTP_ADASAEBReq_enum) -> bus_creator/580
  bus_selector3/1 -> outpmodule/170(VBCM_HornCtrl_flg)  "<VBCM_HornCtrl_flg>"
  bus_selector2/153 -> outpmodule/160(VAPM_DriverSeatBeltCmdTimeOut_flg)  "<VAPM_DriverSeatBeltCmdTimeOut_flg>"
  bus_selector2/151 -> outpmodule/158(VAPM_TCSActiveTimeOut_flg)  "<VAPM_TCSActiveTimeOut_flg>"
  bus_selector16/95 -> outpmodule/644(VVMC_CCMSASpdWar_flg)  "<VVMC_CCMSASpdWar_flg>"
  outpmodule/599(VOUTP_LeftTurnLightReq_flg) -> bus_creator/599
  bus_selector2/149 -> outpmodule/156(VAPM_ABSActiveTimeOut_flg)  "<VAPM_ABSActiveTimeOut_flg>"
  outpmodule/279(VOUTP_HSAFailed_flg) -> bus_creator/279
  outpmodule/413(VOUTP_TPMSCaliButtAllow_flg) -> bus_creator/413
  bus_selector3/4 -> outpmodule/173(VBCM_FROpenClosePBCmd_enum)  "<VBCM_FROpenClosePBCmd_enum>"
  bus_selector2/144 -> outpmodule/151(VAPM_CAASSw_enum)  "<VAPM_CAASSw_enum>"
  outpmodule/456(VOUTP_Chkfin_flg) -> bus_creator/456
  bus_selector2/152 -> outpmodule/159(VAPM_DriverSeatBeltCmd_flg)  "<VAPM_DriverSeatBeltCmd_flg>"
  bus_selector2/143 -> outpmodule/150(VAPM_IVIStatusTimeOut_flg)  "<VAPM_IVIStatusTimeOut_flg>"
  bus_creator/1 -> BOUTP_outputs/1
  bus_selector2/140 -> outpmodule/147(VAPM_AVMErrSTA_flg)  "<VAPM_AVMErrSTA_flg>"
  bus_selector16/83 -> outpmodule/632(VVMC_FCMLDWRequest_enum)  "<VVMC_FCMLDWRequest_enum>"
  bus_selector2/148 -> outpmodule/155(VAPM_ABSActiveToAPM_flg)  "<VAPM_ABSActiveToAPM_flg>"
  bus_selector16/93 -> outpmodule/642(VVMC_APSDecReq_mps2)  "<VVMC_APSDecReq_mps2>"
  bus_selector5/2 -> outpmodule/210(VDKC_DKCAuthSta_enum)  "<VDKC_DKCAuthSta_enum>"
  outpmodule/113(VOUTP_LongAccel_Gps) -> bus_creator/113
  outpmodule/155(VOUTP_ABSActiveToAPM_flg) -> bus_creator/155
  outpmodule/235(VOUTP_HVSysReadyToCharge_enum) -> bus_creator/235
  outpmodule/154(VOUTP_IVIScreenTimeOut_flg) -> bus_creator/154
  outpmodule/153(VOUTP_IVIScreen_enum) -> bus_creator/153
  outpmodule/152(VOUTP_CAASSwTimeOut_flg) -> bus_creator/152
  outpmodule/151(VOUTP_CAASSw_enum) -> bus_creator/151
  outpmodule/149(VOUTP_IVIStatus_flg) -> bus_creator/149
  outpmodule/577(VOUTP_LKAStrToqReq_Nm) -> bus_creator/577
  outpmodule/226(VOUTP_NetworkReq_flg) -> bus_creator/226
  outpmodule/148(VOUTP_AVMErrSTATimeOut_flg) -> bus_creator/148
  bus_selector2/85 -> outpmodule/92(VAPM_ShifterHandleCmdTimeOut_flg)  "<VAPM_ShifterHandleCmdTimeOut_flg>"
  outpmodule/147(VOUTP_AVMErrSTA_flg) -> bus_creator/147
  outpmodule/146(VOUTP_AVMParkingmodeTimeOut_flg) -> bus_creator/146
  outpmodule/144(VOUTP_AVMparkingexcuteTimeOut_flg) -> bus_creator/144
  outpmodule/143(VOUTP_AVMparkingexcute_enum) -> bus_creator/143
  bus_selector2/26 -> outpmodule/33(VAPM_USSStaRMR_flg)  "<VAPM_USSStaRMR_flg>"
  outpmodule/142(VOUTP_AVMparkingcancelTimeOut_flg) -> bus_creator/142
  outpmodule/299(VOUTP_DTbyte3_raw) -> bus_creator/299
  outpmodule/141(VOUTP_AVMparkingcancel_enum) -> bus_creator/141
  outpmodule/358(VOUTP_FDBlowerCmd_pct) -> bus_creator/358
  outpmodule/393(VOUTP_RFBatWarn_flg) -> bus_creator/393
  outpmodule/140(VOUTP_EPBStaTimeOut_flg) -> bus_creator/140
  bus_selector3/19 -> outpmodule/188(VBCM_TurnLpLActiveCmd_flg)  "<VBCM_TurnLpLActiveCmd_flg>"
  outpmodule/139(VOUTP_EPBSta_enum) -> bus_creator/139
  outpmodule/138(VOUTP_EPBErrStaTimeOut_flg) -> bus_creator/138
  outpmodule/137(VOUTP_EPBErrSta_enum) -> bus_creator/137
  outpmodule/457(VOUTP_SetIDLoc_flg) -> bus_creator/457
  outpmodule/136(VOUTP_EPBExtApplyAvailTimeOut_flg) -> bus_creator/136
  outpmodule/134(VOUTP_EPBExtReleaseAvailTimeOut_flg) -> bus_creator/134
  outpmodule/157(VOUTP_TCSActiveToAPM_flg) -> bus_creator/157
  outpmodule/131(VOUTP_ESCAPSSta_enum) -> bus_creator/131
  outpmodule/132(VOUTP_ESCAPSStaTimeOut_flg) -> bus_creator/132
  bus_selector2/114 -> outpmodule/121(VAPM_LongAccelV_flg)  "<VAPM_LongAccelV_flg>"
  outpmodule/308(VOUTP_CarModel2_cnt) -> bus_creator/308
  outpmodule/130(VOUTP_ESCStandstillTimeOut_flg) -> bus_creator/130
  outpmodule/233(VOUTP_DCDCVoltSetpoint_V) -> bus_creator/233
  outpmodule/129(VOUTP_ESCStandstill_flg) -> bus_creator/129
  outpmodule/128(VOUTP_BrkSwVTimeOut_flg) -> bus_creator/128
  outpmodule/125(VOUTP_BrkSwSta_flg) -> bus_creator/125
  bus_selector2/146 -> outpmodule/153(VAPM_IVIScreen_enum)  "<VAPM_IVIScreen_enum>"
  outpmodule/120(VOUTP_LatAccelVTimeOut_flg) -> bus_creator/120
  outpmodule/201(VOUTP_TgateSWRSta_flg) -> bus_creator/201
  bus_selector12/43 -> outpmodule/434(VTPM_S2ID_raw32)  "<VTPM_S2ID_raw32>"
  bus_selector12/38 -> outpmodule/429(VTPM_LFSensorMode_flg)  "<VTPM_LFSensorMode_flg>"
  bus_selector12/35 -> outpmodule/426(VTPM_RRWheelPSW_raw8)  "<VTPM_RRWheelPSW_raw8>"
  outpmodule/464(VOUTP_RRPindi_enum) -> bus_creator/464
  bus_selector12/32 -> outpmodule/423(VTPM_LFWheelPSW_raw8)  "<VTPM_LFWheelPSW_raw8>"
  bus_selector1/2 -> outpmodule/2(VACC_LVBattVoltSta_enum)  "<VACC_LVBattVoltSta_enum>"
  bus_selector12/33 -> outpmodule/424(VTPM_LRWheelPSW_raw8)  "<VTPM_LRWheelPSW_raw8>"
  outpmodule/150(VOUTP_IVIStatusTimeOut_flg) -> bus_creator/150
  bus_selector12/31 -> outpmodule/422(VTPM_RRWheelTmpIndi_flg)  "<VTPM_RRWheelTmpIndi_flg>"
  bus_selector12/34 -> outpmodule/425(VTPM_RFWheelPSW_raw8)  "<VTPM_RFWheelPSW_raw8>"
  bus_selector12/29 -> outpmodule/420(VTPM_RFWheelTmpIndi_flg)  "<VTPM_RFWheelTmpIndi_flg>"
  outpmodule/528(VOUTP_DrvDemEMRtapTrq_pct) -> bus_creator/528
  bus_selector12/25 -> outpmodule/416(VTPM_LRPressIndi_enum)  "<VTPM_LRPressIndi_enum>"
  bus_selector12/26 -> outpmodule/417(VTPM_RRPressIndi_enum)  "<VTPM_RRPressIndi_enum>"
  outpmodule/38(VOUTP_USSStaRCL_flg) -> bus_creator/38
  bus_selector12/24 -> outpmodule/415(VTPM_RFPressIndi_enum)  "<VTPM_RFPressIndi_enum>"
  bus_selector3/22 -> outpmodule/191(VBCM_FrWiperL_flg)  "<VBCM_FrWiperL_flg>"
  outpmodule/493(VOUTP_FrRgnDecrSta_flg) -> bus_creator/493
  bus_selector12/22 -> outpmodule/413(VTPM_TPMSCaliButtAllow_flg)  "<VTPM_TPMSCaliButtAllow_flg>"
  outpmodule/499(VOUTP_FrEDURolRgnTq_Nm) -> bus_creator/499
  bus_selector12/19 -> outpmodule/410(VTPM_RFWheelDebug_flg)  "<VTPM_RFWheelDebug_flg>"
  bus_selector12/20 -> outpmodule/411(VTPM_RRWheelDebug_flg)  "<VTPM_RRWheelDebug_flg>"
  bus_selector12/18 -> outpmodule/409(VTPM_LRWheelDebug_flg)  "<VTPM_LRWheelDebug_flg>"
  outpmodule/500(VOUTP_RrEDURolRgnTq_Nm) -> bus_creator/500
  outpmodule/422(VOUTP_RRWheelTmpIndi_flg) -> bus_creator/422
  bus_selector12/16 -> outpmodule/407(VTPM_RRSensorFail_flg)  "<VTPM_RRSensorFail_flg>"
  bus_selector12/12 -> outpmodule/403(VTPM_RRWheelTemp_C)  "<VTPM_RRWheelTemp_C>"
  outpmodule/2(VOUTP_LVBattVoltSta_enum) -> bus_creator/2
  bus_selector12/7 -> outpmodule/398(VTPM_LRWheelPress_raw8)  "<VTPM_LRWheelPress_raw8>"
  outpmodule/117(VOUTP_YawRateV_flg) -> bus_creator/117
  outpmodule/644(VOUTP_CCMSASpdWar_flg) -> bus_creator/644
  bus_selector12/9 -> outpmodule/400(VTPM_LFWheelTemp_C)  "<VTPM_LFWheelTemp_C>"
  bus_selector2/139 -> outpmodule/146(VAPM_AVMParkingmodeTimeOut_flg)  "<VAPM_AVMParkingmodeTimeOut_flg>"
  bus_selector12/6 -> outpmodule/397(VTPM_RFWheelPress_raw8)  "<VTPM_RFWheelPress_raw8>"
  bus_selector2/102 -> outpmodule/109(VAPM_YawRate_degps)  "<VAPM_YawRate_degps>"
  bus_selector12/5 -> outpmodule/396(VTPM_LFWheelPress_raw8)  "<VTPM_LFWheelPress_raw8>"
  bus_selector11/52 -> outpmodule/391(VTHC_FDCTHCMAPTCWarningSta_flg)  "<VTHC_FDCTHCMAPTCWarningSta_flg>"
  outpmodule/104(VOUTP_SASCALTimeOut_flg) -> bus_creator/104
  outpmodule/341(VOUTP_FDSOV1Cmd_flg) -> bus_creator/341
  bus_selector11/50 -> outpmodule/389(VTHC_fdefog_flg)  "<VTHC_fdefog_flg>"
  bus_selector11/47 -> outpmodule/386(VTHC_ACForceOFF_flg)  "<VTHC_ACForceOFF_flg>"
  bus_selector11/44 -> outpmodule/383(VTHC_FaceM_flg)  "<VTHC_FaceM_flg>"
  outpmodule/135(VOUTP_EPBExtApplyAvail_flg) -> bus_creator/135
  bus_selector3/14 -> outpmodule/183(VBCM_HazardSW_flg)  "<VBCM_HazardSW_flg>"
  bus_selector2/76 -> outpmodule/83(VAPM_LFPulseCount_enum)  "<VAPM_LFPulseCount_enum>"
  outpmodule/640(VOUTP_APSStaSys_enum) -> bus_creator/640
  bus_selector11/45 -> outpmodule/384(VTHC_FootM_flg)  "<VTHC_FootM_flg>"
  bus_selector2/159 -> outpmodule/166(VAPM_APSAngleTarget_Deg)  "<VAPM_APSAngleTarget_Deg>"
  bus_selector11/43 -> outpmodule/382(VTHC_Frost_flg)  "<VTHC_Frost_flg>"
  outpmodule/462(VOUTP_RFPind_enum) -> bus_creator/462
  outpmodule/426(VOUTP_RRWheelPSW_raw8) -> bus_creator/426
  bus_selector11/39 -> outpmodule/378(VTHC_FDRecyAutoCmd_enum)  "<VTHC_FDRecyAutoCmd_enum>"
  BAPM_outputs/1 -> bus_selector2/1
  bus_selector11/37 -> outpmodule/376(VTHC_sigCbnAirT_C)  "<VTHC_sigCbnAirT_C>"
  bus_selector16/96 -> outpmodule/645(VVMC_IMUEnaCmd_flg)  "<VVMC_IMUEnaCmd_flg>"
  outpmodule/454(VOUTP_ID3messageALTU_raw8) -> bus_creator/454
  bus_selector12/37 -> outpmodule/428(VTPM_AutoLTips_enum)  "<VTPM_AutoLTips_enum>"
  bus_selector11/38 -> outpmodule/377(VTHC_ACSubMode_enum)  "<VTHC_ACSubMode_enum>"
  bus_selector11/36 -> outpmodule/375(VTHC_sigAmbAirT_C)  "<VTHC_sigAmbAirT_C>"
  bus_selector12/46 -> outpmodule/437(VTPM_S1L_enum)  "<VTPM_S1L_enum>"
  outpmodule/628(VOUTP_ADASLanetypeL_enum) -> bus_creator/628
  bus_selector1/7 -> outpmodule/7(VACC_EACEnDem_enum)  "<VACC_EACEnDem_enum>"
  outpmodule/630(VOUTP_ADASLanecurveR_raw32) -> bus_creator/630
  outpmodule/629(VOUTP_ADASLanecurveL_raw32) -> bus_creator/629
  outpmodule/121(VOUTP_LongAccelV_flg) -> bus_creator/121
  outpmodule/626(VOUTP_FCMACCmode_enum) -> bus_creator/626
  outpmodule/254(VOUTP_IVIPwrStaONTOPopT_s) -> bus_creator/254
  outpmodule/624(VOUTP_LVDAACCStatusInformation_flg) -> bus_creator/624
  outpmodule/621(VOUTP_LVDAMuteSta_enum) -> bus_creator/621
  bus_selector2/155 -> outpmodule/162(VAPM_APSRQDisplay_enum)  "<VAPM_APSRQDisplay_enum>"
  outpmodule/618(VOUTP_ADASFCWMute_flg) -> bus_creator/618
  outpmodule/612(VOUTP_ADASLFCSta_enum) -> bus_creator/612
  outpmodule/608(VOUTP_TargetType_enum) -> bus_creator/608
  outpmodule/552(VOUTP_VehicleSpeed_kph) -> bus_creator/552
  outpmodule/607(VOUTP_ADASCAMSpdLim_enum) -> bus_creator/607
  outpmodule/605(VOUTP_ACCTakeoverReq_flg) -> bus_creator/605
  BDHP_outputs/1 -> bus_selector4/1
  outpmodule/231(VOUTP_ActiveDischargeReq_flg) -> bus_creator/231
  outpmodule/633(VOUTP_FCMLDWFault_flg) -> bus_creator/633
  outpmodule/277(VOUTP_AmberWnlmpSta_flg) -> bus_creator/277
  bus_selector12/17 -> outpmodule/408(VTPM_LFWheelDebug_flg)  "<VTPM_LFWheelDebug_flg>"
  BTQR_outputs/1 -> bus_selector14/1
  outpmodule/561(VOUTP_LimitPCT_pct) -> bus_creator/561
  bus_selector14/2 -> outpmodule/547(VTQR_RrTMTqReq_Nm)  "<VTQR_RrTMTqReq_Nm>"
  bus_selector12/30 -> outpmodule/421(VTPM_LRWheelTmpIndi_flg)  "<VTPM_LRWheelTmpIndi_flg>"
  bus_selector2/141 -> outpmodule/148(VAPM_AVMErrSTATimeOut_flg)  "<VAPM_AVMErrSTATimeOut_flg>"
  bus_selector14/1 -> outpmodule/546(VTQR_FrTMTqReq_Nm)  "<VTQR_FrTMTqReq_Nm>"
  bus_selector2/42 -> outpmodule/49(VAPM_BrkPedalPosToAPM_pct)  "<VAPM_BrkPedalPosToAPM_pct>"
  BTQD_outputs/1 -> bus_selector13/1
  bus_selector13/63 -> outpmodule/545(VTQD_FDCVCUDACStatusSta_enum)  "<VTQD_FDCVCUDACStatusSta_enum>"
  bus_selector13/61 -> outpmodule/543(VTQD_FDCCHAEBSHHSwSta_enum)  "<VTQD_FDCCHAEBSHHSwSta_enum>"
  outpmodule/484(VOUTP_TqSourceFr_enum) -> bus_creator/484
  bus_selector10/28 -> outpmodule/331(VSYS_SHA7_cnt)  "<VSYS_SHA7_cnt>"
  outpmodule/390(VOUTP_sigSetTempZon2StM_C) -> bus_creator/390
  bus_selector13/60 -> outpmodule/542(VTQD_FDCCHAEBSHBSwSta_enum)  "<VTQD_FDCCHAEBSHBSwSta_enum>"
  bus_selector12/15 -> outpmodule/406(VTPM_LRSensorFail_flg)  "<VTPM_LRSensorFail_flg>"
  bus_selector13/57 -> outpmodule/539(VTQD_EEC2MSGCnt_raw)  "<VTQD_EEC2MSGCnt_raw>"
  bus_selector12/1 -> outpmodule/392(VTPM_LFBatWarn_flg)  "<VTPM_LFBatWarn_flg>"
  outpmodule/107(VOUTP_GRADE_Deg) -> bus_creator/107
  bus_selector13/56 -> outpmodule/538(VTQD_EMParasLoss_pct)  "<VTQD_EMParasLoss_pct>"
  outpmodule/363(VOUTP_CCUAutoLampSts_flg) -> bus_creator/363
  bus_selector2/150 -> outpmodule/157(VAPM_TCSActiveToAPM_flg)  "<VAPM_TCSActiveToAPM_flg>"
  bus_selector13/59 -> outpmodule/541(VTQD_FDCCHAEBSRd4BRSta_enum)  "<VTQD_FDCCHAEBSRd4BRSta_enum>"
  bus_selector13/51 -> outpmodule/533(VTQD_AccPedalPos1_pct)  "<VTQD_AccPedalPos1_pct>"
  outpmodule/348(VOUTP_FDTWVCmd_pct) -> bus_creator/348
  outpmodule/455(VOUTP_ID4messageALTU_raw8) -> bus_creator/455
  outpmodule/283(VOUTP_HSAActive_flg) -> bus_creator/283
  outpmodule/545(VOUTP_FDCVCUDACStatusSta_enum) -> bus_creator/545
  bus_selector13/52 -> outpmodule/534(VTQD_ParkBrakeSW_enum)  "<VTQD_ParkBrakeSW_enum>"
  bus_selector12/28 -> outpmodule/419(VTPM_LFWheelTmpIndi_flg)  "<VTPM_LFWheelTmpIndi_flg>"
  bus_selector13/49 -> outpmodule/531(VTQD_ShiftPgs_enum)  "<VTQD_ShiftPgs_enum>"
  outpmodule/508(VOUTP_PTCSPermSta_flg) -> bus_creator/508
  outpmodule/425(VOUTP_RFWheelPSW_raw8) -> bus_creator/425
  bus_selector13/50 -> outpmodule/532(VTQD_AccPedal1LowSW_enum)  "<VTQD_AccPedal1LowSW_enum>"
  bus_selector13/45 -> outpmodule/527(VTQD_ActEMOutSftSpd_rpm)  "<VTQD_ActEMOutSftSpd_rpm>"
  bus_selector2/78 -> outpmodule/85(VAPM_RFPulseCount_enum)  "<VAPM_RFPulseCount_enum>"
  bus_selector13/44 -> outpmodule/526(VTQD_ActEMpTrqHrls_pct)  "<VTQD_ActEMpTrqHrls_pct>"
  bus_selector3/21 -> outpmodule/190(VBCM_BBuzzerCmd_flg)  "<VBCM_BBuzzerCmd_flg>"
  outpmodule/460(VOUTP_TPMSResButt_flg) -> bus_creator/460
  outpmodule/396(VOUTP_LFWheelPress_raw8) -> bus_creator/396
  bus_selector13/43 -> outpmodule/525(VTQD_EMTrqModeDrvBrk_enum)  "<VTQD_EMTrqModeDrvBrk_enum>"
  bus_selector12/44 -> outpmodule/435(VTPM_S3ID_raw32)  "<VTPM_S3ID_raw32>"
  bus_selector13/42 -> outpmodule/524(VTQD_DLEngaged_enum)  "<VTQD_DLEngaged_enum>"
  bus_selector13/40 -> outpmodule/522(VTQD_ActMaxAvaEMRecpTrq_pct)  "<VTQD_ActMaxAvaEMRecpTrq_pct>"
  bus_selector13/38 -> outpmodule/520(VTQD_CreepON_flg)  "<VTQD_CreepON_flg>"
  outpmodule/513(VOUTP_FrUdcMin_V) -> bus_creator/513
  bus_selector2/135 -> outpmodule/142(VAPM_AVMparkingcancelTimeOut_flg)  "<VAPM_AVMparkingcancelTimeOut_flg>"
  bus_selector12/27 -> outpmodule/418(VTPM_TPMSWarnIndi_enum)  "<VTPM_TPMSWarnIndi_enum>"
  bus_selector13/36 -> outpmodule/518(VTQD_RrUdcMax_V)  "<VTQD_RrUdcMax_V>"
  bus_selector2/156 -> outpmodule/163(VAPM_APSSWVer_enum)  "<VAPM_APSSWVer_enum>"
  bus_selector13/39 -> outpmodule/521(VTQD_ActEMpTrq_pct)  "<VTQD_ActEMpTrq_pct>"
  bus_selector3/5 -> outpmodule/174(VBCM_DoorStaSta_enum)  "<VBCM_DoorStaSta_enum>"
  bus_selector13/35 -> outpmodule/517(VTQD_RrUdcMin_V)  "<VTQD_RrUdcMin_V>"
  outpmodule/453(VOUTP_ID2messageALTU_raw8) -> bus_creator/453
  bus_selector16/18 -> outpmodule/567(VVMC_SPD2ACCAct_flg)  "<VVMC_SPD2ACCAct_flg>"
  bus_selector16/15 -> outpmodule/564(VVMC_SingleWhlSlipRatioCtrl_flg)  "<VVMC_SingleWhlSlipRatioCtrl_flg>"
  bus_selector3/10 -> outpmodule/179(VBCM_RrFogLamp_flg)  "<VBCM_RrFogLamp_flg>"
  bus_selector16/13 -> outpmodule/562(VVMC_FrontRearSlipRatioCtrl_flg)  "<VVMC_FrontRearSlipRatioCtrl_flg>"
  bus_selector12/42 -> outpmodule/433(VTPM_S1ID_raw32)  "<VTPM_S1ID_raw32>"
  bus_selector16/14 -> outpmodule/563(VVMC_RearWhlSlipRatioCtrl_flg)  "<VVMC_RearWhlSlipRatioCtrl_flg>"
  bus_selector11/46 -> outpmodule/385(VTHC_CCUSyncSts_flg)  "<VTHC_CCUSyncSts_flg>"
  bus_selector16/10 -> outpmodule/559(VVMC_FeatReqSpd_kph)  "<VVMC_FeatReqSpd_kph>"
  bus_selector12/41 -> outpmodule/432(VTPM_RRSensorMode_flg)  "<VTPM_RRSensorMode_flg>"
  outpmodule/428(VOUTP_AutoLTips_enum) -> bus_creator/428
  bus_selector16/8 -> outpmodule/557(VVMC_VMCMSACtrlAvail_flg)  "<VVMC_VMCMSACtrlAvail_flg>"
  outpmodule/568(VOUTP_AccCalcuPID_mps2) -> bus_creator/568
  outpmodule/242(VOUTP_DrivetrainSelect_enum) -> bus_creator/242
  bus_selector16/11 -> outpmodule/560(VVMC_JerkPCT_pct)  "<VVMC_JerkPCT_pct>"
  bus_selector12/8 -> outpmodule/399(VTPM_RRWheelPress_raw8)  "<VTPM_RRWheelPress_raw8>"
  outpmodule/468(VOUTP_WriteChkRRID_raw) -> bus_creator/468
  outpmodule/616(VOUTP_ADASISASta_enum) -> bus_creator/616
  bus_selector16/7 -> outpmodule/556(VVMC_VMCCCCtrlAvail_flg)  "<VVMC_VMCCCCtrlAvail_flg>"
  bus_selector12/23 -> outpmodule/414(VTPM_LFPressIndi_enum)  "<VTPM_LFPressIndi_enum>"
  bus_selector2/137 -> outpmodule/144(VAPM_AVMparkingexcuteTimeOut_flg)  "<VAPM_AVMparkingexcuteTimeOut_flg>"
  bus_selector3/3 -> outpmodule/172(VBCM_FRDisIntEmCmd_flg)  "<VBCM_FRDisIntEmCmd_flg>"
  bus_selector16/3 -> outpmodule/552(VVMC_VehicleSpeed_kph)  "<VVMC_VehicleSpeed_kph>"
  BV2L_outputs/1 -> bus_selector15/1
  outpmodule/556(VOUTP_VMCCCCtrlAvail_flg) -> bus_creator/556
  outpmodule/219(VOUTP_ErrorState_enum) -> bus_creator/219
  bus_selector12/2 -> outpmodule/393(VTPM_RFBatWarn_flg)  "<VTPM_RFBatWarn_flg>"
  outpmodule/582(VOUTP_AEBVehHoldReq_flg) -> bus_creator/582
  bus_selector16/1 -> outpmodule/550(VVMC_FeatSetSpdFinal_raw32)  "<VVMC_FeatSetSpdFinal_raw32>"
  outpmodule/405(VOUTP_RFSensorFail_flg) -> bus_creator/405
  bus_selector16/36 -> outpmodule/585(VVMC_ADASACCSta_enum)  "<VVMC_ADASACCSta_enum>"
  bus_selector13/6 -> outpmodule/488(VTQD_EVDriveMode_enum)  "<VTQD_EVDriveMode_enum>"
  bus_selector13/7 -> outpmodule/489(VTQD_ShiftGearPosn_enum)  "<VTQD_ShiftGearPosn_enum>"
  bus_selector13/5 -> outpmodule/487(VTQD_RrEDUAvailBrkRgnTq_Nm)  "<VTQD_RrEDUAvailBrkRgnTq_Nm>"
  outpmodule/530(VOUTP_RetSelNonEng_pct) -> bus_creator/530
  bus_selector13/2 -> outpmodule/484(VTQD_TqSourceFr_enum)  "<VTQD_TqSourceFr_enum>"
  bus_selector16/24 -> outpmodule/573(VVMC_DISCReqAcc_mps2)  "<VVMC_DISCReqAcc_mps2>"
  bus_selector12/90 -> outpmodule/481(VTPM_FlashS4ID_raw)  "<VTPM_FlashS4ID_raw>"
  bus_selector12/91 -> outpmodule/482(VTPM_FlashIDvalid_enum)  "<VTPM_FlashIDvalid_enum>"
  bus_selector12/88 -> outpmodule/479(VTPM_FlashS2ID_raw)  "<VTPM_FlashS2ID_raw>"
  outpmodule/116(VOUTP_MCPressureTimeOut_flg) -> bus_creator/116
  outpmodule/529(VOUTP_SACtrlDev_enum) -> bus_creator/529
  bus_selector12/86 -> outpmodule/477(VTPM_Prepresstempvalid_enum)  "<VTPM_Prepresstempvalid_enum>"
  bus_selector16/43 -> outpmodule/592(VVMC_ACCComfortBandLower_mps2)  "<VVMC_ACCComfortBandLower_mps2>"
  bus_selector12/87 -> outpmodule/478(VTPM_FlashS1ID_raw)  "<VTPM_FlashS1ID_raw>"
  bus_selector2/154 -> outpmodule/161(VAPM_APSProgressPCT_pct)  "<VAPM_APSProgressPCT_pct>"
  bus_selector12/84 -> outpmodule/475(VTPM_unlearnSfali_flg)  "<VTPM_unlearnSfali_flg>"
  bus_selector12/85 -> outpmodule/476(VTPM_unlearnSfailvalid_enum)  "<VTPM_unlearnSfailvalid_enum>"
  outpmodule/461(VOUTP_LFPindi_enum) -> bus_creator/461
  bus_selector12/80 -> outpmodule/471(VTPM_WriteChkfinLRID_raw)  "<VTPM_WriteChkfinLRID_raw>"
  outpmodule/8(VOUTP_VehSpeedToAPM_kph) -> bus_creator/8
  outpmodule/571(VOUTP_ISOJerkLimit_mps3) -> bus_creator/571
  bus_selector12/79 -> outpmodule/470(VTPM_WriteChkfinRFID_raw)  "<VTPM_WriteChkfinRFID_raw>"
  bus_selector3/12 -> outpmodule/181(VBCM_LBeam_flg)  "<VBCM_LBeam_flg>"
  outpmodule/211(VOUTP_DISCTurn_flg) -> bus_creator/211
  bus_selector13/37 -> outpmodule/519(VTQD_ReBrakeLPReq_flg)  "<VTQD_ReBrakeLPReq_flg>"
  outpmodule/349(VOUTP_FDFrWPTCHeatPwrCmd_W) -> bus_creator/349
  bus_selector12/78 -> outpmodule/469(VTPM_WriteChkfinLFID_raw)  "<VTPM_WriteChkfinLFID_raw>"
  outpmodule/52(VOUTP_LFRawWhlSpeedTimeOut_flg) -> bus_creator/52
  outpmodule/322(VOUTP_Change1_cnt) -> bus_creator/322
  bus_selector16/75 -> outpmodule/624(VVMC_LVDAACCStatusInformation_flg)  "<VVMC_LVDAACCStatusInformation_flg>"
  bus_selector12/77 -> outpmodule/468(VTPM_WriteChkRRID_raw)  "<VTPM_WriteChkRRID_raw>"
  bus_selector10/12 -> outpmodule/315(VSYS_Minor2_cnt)  "<VSYS_Minor2_cnt>"
  bus_selector12/76 -> outpmodule/467(VTPM_WriteChkLRID_raw)  "<VTPM_WriteChkLRID_raw>"
  bus_selector3/16 -> outpmodule/185(VBCM_RTurnLP_flg)  "<VBCM_RTurnLP_flg>"
  outpmodule/95(VOUTP_EPSAOIControl_enum) -> bus_creator/95
  outpmodule/338(VOUTP_AcoreRebootCmdACK_flg) -> bus_creator/338
  outpmodule/80(VOUTP_LRPulseCountVTimeOut_flg) -> bus_creator/80
  bus_selector2/60 -> outpmodule/67(VAPM_LFWhlRotDir_enum)  "<VAPM_LFWhlRotDir_enum>"
  bus_selector12/75 -> outpmodule/466(VTPM_WriteChkRFID_raw)  "<VTPM_WriteChkRFID_raw>"
  bus_selector2/161 -> outpmodule/168(VAPM_APSRqEPASCtrl_flg)  "<VAPM_APSRqEPASCtrl_flg>"
  outpmodule/102(VOUTP_SASSpeedValidTimeOut_flg) -> bus_creator/102
  BTHC_outputs/1 -> bus_selector11/1
  bus_selector12/74 -> outpmodule/465(VTPM_WriteChkLFID_raw)  "<VTPM_WriteChkLFID_raw>"
  bus_selector2/160 -> outpmodule/167(VAPM_APSVRqEPASCtrl_flg)  "<VAPM_APSVRqEPASCtrl_flg>"
  bus_selector12/73 -> outpmodule/464(VTPM_RRPindi_enum)  "<VTPM_RRPindi_enum>"
  outpmodule/89(VOUTP_RRPulseCount_enum) -> bus_creator/89
  bus_selector16/16 -> outpmodule/565(VVMC_LatAccCtrl_flg)  "<VVMC_LatAccCtrl_flg>"
  bus_selector12/72 -> outpmodule/463(VTPM_LRPindi_enum)  "<VTPM_LRPindi_enum>"
  outpmodule/85(VOUTP_RFPulseCount_enum) -> bus_creator/85
  bus_selector12/70 -> outpmodule/461(VTPM_LFPindi_enum)  "<VTPM_LFPindi_enum>"
  bus_selector12/71 -> outpmodule/462(VTPM_RFPind_enum)  "<VTPM_RFPind_enum>"
  bus_selector12/67 -> outpmodule/458(VTPM_TPMSStorge_flg)  "<VTPM_TPMSStorge_flg>"
  outpmodule/523(VOUTP_ActDriveDirect_enum) -> bus_creator/523
  bus_selector16/54 -> outpmodule/603(VVMC_ACCObjDstLvl_enum)  "<VVMC_ACCObjDstLvl_enum>"
  bus_selector12/68 -> outpmodule/459(VTPM_ChkStorge_flg)  "<VTPM_ChkStorge_flg>"
  outpmodule/622(VOUTP_LVDAFailinfo_flg) -> bus_creator/622
  bus_selector12/65 -> outpmodule/456(VTPM_Chkfin_flg)  "<VTPM_Chkfin_flg>"
  bus_selector12/66 -> outpmodule/457(VTPM_SetIDLoc_flg)  "<VTPM_SetIDLoc_flg>"
  outpmodule/199(VOUTP_TgateHDSWRSta_flg) -> bus_creator/199
  outpmodule/496(VOUTP_DriverWhlTqDemRr_Nm) -> bus_creator/496
  bus_selector12/63 -> outpmodule/454(VTPM_ID3messageALTU_raw8)  "<VTPM_ID3messageALTU_raw8>"
  outpmodule/535(VOUTP_VCUVehSpd_kph) -> bus_creator/535
  bus_selector12/58 -> outpmodule/449(VTPM_S2WheelDebugALTU_pct)  "<VTPM_S2WheelDebugALTU_pct>"
  outpmodule/389(VOUTP_fdefog_flg) -> bus_creator/389
  bus_selector12/57 -> outpmodule/448(VTPM_S1WheelDebugALTU_pct)  "<VTPM_S1WheelDebugALTU_pct>"
  bus_selector2/63 -> outpmodule/70(VAPM_RFWhlRotDirTimeOut_flg)  "<VAPM_RFWhlRotDirTimeOut_flg>"
  bus_selector3/17 -> outpmodule/186(VBCM_LSMLPCmd_flg)  "<VBCM_LSMLPCmd_flg>"
  bus_selector12/56 -> outpmodule/447(VTPM_IDin_raw32)  "<VTPM_IDin_raw32>"
  bus_selector16/70 -> outpmodule/619(VVMC_ADASLFCHandsOffWarning_enum)  "<VVMC_ADASLFCHandsOffWarning_enum>"
  bus_selector12/53 -> outpmodule/444(VTPM_LRP20_raw8)  "<VTPM_LRP20_raw8>"
  bus_selector11/51 -> outpmodule/390(VTHC_sigSetTempZon2StM_C)  "<VTHC_sigSetTempZon2StM_C>"
  outpmodule/247(VOUTP_PwrUpReq_enum) -> bus_creator/247
  bus_selector12/55 -> outpmodule/446(VTPM_FAT_flg)  "<VTPM_FAT_flg>"
  bus_selector12/54 -> outpmodule/445(VTPM_RRP20_raw8)  "<VTPM_RRP20_raw8>"
  outpmodule/441(VOUTP_ALFin_flg) -> bus_creator/441
  bus_selector16/6 -> outpmodule/555(VVMC_VMCACCCtrlAvail_flg)  "<VVMC_VMCACCCtrlAvail_flg>"
  bus_selector16/60 -> outpmodule/609(VVMC_ADASSLIFSpdLim_enum)  "<VVMC_ADASSLIFSpdLim_enum>"
  bus_selector12/52 -> outpmodule/443(VTPM_RFP20_raw8)  "<VTPM_RFP20_raw8>"
  bus_selector12/51 -> outpmodule/442(VTPM_LFP20_raw8)  "<VTPM_LFP20_raw8>"
  bus_selector13/33 -> outpmodule/515(VTQD_RrIdcMin_A)  "<VTQD_RrIdcMin_A>"
  bus_selector16/17 -> outpmodule/566(VVMC_SafetyCtrl_flg)  "<VVMC_SafetyCtrl_flg>"
  outpmodule/334(VOUTP_FdcSlpReqRisingEdge_flg) -> bus_creator/334
  bus_selector3/36 -> outpmodule/205(VBCM_FDDoorstate_enum)  "<VBCM_FDDoorstate_enum>"
  outpmodule/541(VOUTP_FDCCHAEBSRd4BRSta_enum) -> bus_creator/541
  outpmodule/20(VOUTP_PASDFCL_cm) -> bus_creator/20
  bus_selector13/32 -> outpmodule/514(VTQD_FrUdcMax_V)  "<VTQD_FrUdcMax_V>"
  outpmodule/512(VOUTP_FrIdcMax_A) -> bus_creator/512
  bus_selector3/2 -> outpmodule/171(VBCM_FRHaltBrakeSta_enum)  "<VBCM_FRHaltBrakeSta_enum>"
  bus_selector13/30 -> outpmodule/512(VTQD_FrIdcMax_A)  "<VTQD_FrIdcMax_A>"
  bus_selector2/55 -> outpmodule/62(VAPM_RFRawWhlSpeedVTimeOut_flg)  "<VAPM_RFRawWhlSpeedVTimeOut_flg>"
  bus_selector13/31 -> outpmodule/513(VTQD_FrUdcMin_V)  "<VTQD_FrUdcMin_V>"
  outpmodule/601(VOUTP_ADASLDWSta_enum) -> bus_creator/601
  outpmodule/115(VOUTP_MCPressure_bar) -> bus_creator/115
  bus_selector16/19 -> outpmodule/568(VVMC_AccCalcuPID_mps2)  "<VVMC_AccCalcuPID_mps2>"
  bus_selector12/81 -> outpmodule/472(VTPM_WriteChkfinRRID_raw)  "<VTPM_WriteChkfinRRID_raw>"
  outpmodule/45(VOUTP_Chime_enum) -> bus_creator/45
  bus_selector13/28 -> outpmodule/510(VTQD_RrRgnPermSta_flg)  "<VTQD_RrRgnPermSta_flg>"
  bus_selector13/24 -> outpmodule/506(VTQD_RrEDUAvailBrkRgnTqV_flg)  "<VTQD_RrEDUAvailBrkRgnTqV_flg>"
  bus_selector13/26 -> outpmodule/508(VTQD_PTCSPermSta_flg)  "<VTQD_PTCSPermSta_flg>"
  bus_selector16/35 -> outpmodule/584(VVMC_ADASDBSReq_enum)  "<VVMC_ADASDBSReq_enum>"
  bus_selector13/25 -> outpmodule/507(VTQD_RgnAbnorSta_flg)  "<VTQD_RgnAbnorSta_flg>"
  outpmodule/100(VOUTP_SASSpeedTimeOut_flg) -> bus_creator/100
  bus_selector13/23 -> outpmodule/505(VTQD_RrEDUSpdValid_flg)  "<VTQD_RrEDUSpdValid_flg>"
  bus_selector13/21 -> outpmodule/503(VTQD_FrEDUSpdValid_flg)  "<VTQD_FrEDUSpdValid_flg>"
  outpmodule/27(VOUTP_PASARML_enum) -> bus_creator/27
  outpmodule/69(VOUTP_RFWhlRotDir_enum) -> bus_creator/69
  outpmodule/395(VOUTP_RRBatWarn_flg) -> bus_creator/395
  bus_selector11/49 -> outpmodule/388(VTHC_AirIntenZone1M_enum)  "<VTHC_AirIntenZone1M_enum>"
  bus_selector13/17 -> outpmodule/499(VTQD_FrEDURolRgnTq_Nm)  "<VTQD_FrEDURolRgnTq_Nm>"
  outpmodule/295(VOUTP_triggerDT_flg) -> bus_creator/295
  bus_selector13/18 -> outpmodule/500(VTQD_RrEDURolRgnTq_Nm)  "<VTQD_RrEDURolRgnTq_Nm>"
  bus_selector11/48 -> outpmodule/387(VTHC_RecAutoFlg_flg)  "<VTHC_RecAutoFlg_flg>"
  bus_selector16/12 -> outpmodule/561(VVMC_LimitPCT_pct)  "<VVMC_LimitPCT_pct>"
  outpmodule/606(VOUTP_ADASWarningMsg_enum) -> bus_creator/606
  outpmodule/638(VOUTP_MSACtrlSta_enum) -> bus_creator/638
  bus_selector2/127 -> outpmodule/134(VAPM_EPBExtReleaseAvailTimeOut_flg)  "<VAPM_EPBExtReleaseAvailTimeOut_flg>"
  bus_selector13/14 -> outpmodule/496(VTQD_DriverWhlTqDemRr_Nm)  "<VTQD_DriverWhlTqDemRr_Nm>"
  outpmodule/293(VOUTP_CFGEM1BAMRsv_raw) -> bus_creator/293
  bus_selector13/16 -> outpmodule/498(VTQD_RrEDUActTq_Nm)  "<VTQD_RrEDUActTq_Nm>"
  bus_selector16/23 -> outpmodule/572(VVMC_ACCRequiredAccel_mps2)  "<VVMC_ACCRequiredAccel_mps2>"
  outpmodule/485(VOUTP_TqSourceRr_enum) -> bus_creator/485
  bus_selector3/7 -> outpmodule/176(VBCM_LDRL_flg)  "<VBCM_LDRL_flg>"
  outpmodule/604(VOUTP_ForceLowBeam_enum) -> bus_creator/604
  bus_selector13/15 -> outpmodule/497(VTQD_FrEDUActTq_Nm)  "<VTQD_FrEDUActTq_Nm>"
  bus_selector13/11 -> outpmodule/493(VTQD_FrRgnDecrSta_flg)  "<VTQD_FrRgnDecrSta_flg>"
  outpmodule/238(VOUTP_HVPwrSta_flg) -> bus_creator/238
  outpmodule/55(VOUTP_LRRawWhlSpeed_kph) -> bus_creator/55
  bus_selector13/12 -> outpmodule/494(VTQD_RrRgnDecrSta_flg)  "<VTQD_RrRgnDecrSta_flg>"
  bus_selector16/2 -> outpmodule/551(VVMC_VehicleSpeed_mph)  "<VVMC_VehicleSpeed_mph>"
  bus_selector11/42 -> outpmodule/381(VTHC_Foot_flg)  "<VTHC_Foot_flg>"
  bus_selector8/20 -> outpmodule/246(VPMM_TCountSta_enum)  "<VPMM_TCountSta_enum>"
  outpmodule/634(VOUTP_ACCCtrlAvail_flg) -> bus_creator/634
  bus_selector8/21 -> outpmodule/247(VPMM_PwrUpReq_enum)  "<VPMM_PwrUpReq_enum>"
  bus_selector8/16 -> outpmodule/242(VPMM_DrivetrainSelect_enum)  "<VPMM_DrivetrainSelect_enum>"
  bus_selector8/14 -> outpmodule/240(VPMM_FrMCUEnaReq_flg)  "<VPMM_FrMCUEnaReq_flg>"
  bus_selector8/11 -> outpmodule/237(VPMM_LVPwrSta_flg)  "<VPMM_LVPwrSta_flg>"
  outpmodule/26(VOUTP_PASARMR_enum) -> bus_creator/26
  outpmodule/488(VOUTP_EVDriveMode_enum) -> bus_creator/488
  bus_selector8/15 -> outpmodule/241(VPMM_RrMCUEnaReq_flg)  "<VPMM_RrMCUEnaReq_flg>"
  outpmodule/145(VOUTP_AVMParkingmode_enum) -> bus_creator/145
  bus_selector8/12 -> outpmodule/238(VPMM_HVPwrSta_flg)  "<VPMM_HVPwrSta_flg>"
  outpmodule/297(VOUTP_DTbyte1_raw) -> bus_creator/297
  bus_selector13/54 -> outpmodule/536(VTQD_BrakeSW_enum)  "<VTQD_BrakeSW_enum>"
  bus_selector1/4 -> outpmodule/4(VACC_EHPSEnDem_enum)  "<VACC_EHPSEnDem_enum>"
  bus_selector8/7 -> outpmodule/233(VPMM_DCDCVoltSetpoint_V)  "<VPMM_DCDCVoltSetpoint_V>"
  outpmodule/191(VOUTP_FrWiperL_flg) -> bus_creator/191
  bus_selector8/13 -> outpmodule/239(VPMM_SysPowerMode_enum)  "<VPMM_SysPowerMode_enum>"
  bus_selector2/142 -> outpmodule/149(VAPM_IVIStatus_flg)  "<VAPM_IVIStatus_flg>"
  outpmodule/202(VOUTP_LTgateRelCmd_flg) -> bus_creator/202
  bus_selector8/8 -> outpmodule/234(VPMM_HVBatCnctReq_flg)  "<VPMM_HVBatCnctReq_flg>"
  bus_selector13/9 -> outpmodule/491(VTQD_FrActvDmpDisabReq_flg)  "<VTQD_FrActvDmpDisabReq_flg>"
  outpmodule/229(VOUTP_PowerUpFault_enum) -> bus_creator/229
  outpmodule/352(VOUTP_FDEWP1Cmd_enum) -> bus_creator/352
  outpmodule/49(VOUTP_BrkPedalPosToAPM_pct) -> bus_creator/49
  bus_selector8/1 -> outpmodule/227(VPMM_PowerUpState_enum)  "<VPMM_PowerUpState_enum>"
  bus_selector16/78 -> outpmodule/627(VVMC_ADASLanetypeR_enum)  "<VVMC_ADASLanetypeR_enum>"
  outpmodule/473(VOUTP_Flashchkdatavalid_enum) -> bus_creator/473
  outpmodule/614(VOUTP_ADASLaneModeR_enum) -> bus_creator/614
  bus_selector8/4 -> outpmodule/230(VPMM_PowerDownFault_enum)  "<VPMM_PowerDownFault_enum>"
  outpmodule/362(VOUTP_CCUACLampSts_flg) -> bus_creator/362
  bus_selector12/14 -> outpmodule/405(VTPM_RFSensorFail_flg)  "<VTPM_RFSensorFail_flg>"
  outpmodule/527(VOUTP_ActEMOutSftSpd_rpm) -> bus_creator/527
  bus_selector8/3 -> outpmodule/229(VPMM_PowerUpFault_enum)  "<VPMM_PowerUpFault_enum>"
  bus_selector8/2 -> outpmodule/228(VPMM_PowerDownState_enum)  "<VPMM_PowerDownState_enum>"
  bus_selector8/5 -> outpmodule/231(VPMM_ActiveDischargeReq_flg)  "<VPMM_ActiveDischargeReq_flg>"
  bus_selector10/6 -> outpmodule/309(VSYS_CarModel3_cnt)  "<VSYS_CarModel3_cnt>"
  outpmodule/161(VOUTP_APSProgressPCT_pct) -> bus_creator/161
  bus_selector10/4 -> outpmodule/307(VSYS_CarModel1_cnt)  "<VSYS_CarModel1_cnt>"
  bus_selector12/61 -> outpmodule/452(VTPM_ID1messageALTU_raw8)  "<VTPM_ID1messageALTU_raw8>"
  bus_selector13/34 -> outpmodule/516(VTQD_RrIdcMax_A)  "<VTQD_RrIdcMax_A>"
  bus_selector10/1 -> outpmodule/304(VSYS_HWVer1_cnt)  "<VSYS_HWVer1_cnt>"
  bus_selector2/62 -> outpmodule/69(VAPM_RFWhlRotDir_enum)  "<VAPM_RFWhlRotDir_enum>"
  bus_selector12/36 -> outpmodule/427(VTPM_CWheelTips_enum)  "<VTPM_CWheelTips_enum>"
  outpmodule/208(VOUTP_EAPS2MIN_pct) -> bus_creator/208
  bus_selector10/3 -> outpmodule/306(VSYS_HWVer3_cnt)  "<VSYS_HWVer3_cnt>"
  outpmodule/542(VOUTP_FDCCHAEBSHBSwSta_enum) -> bus_creator/542
  bus_selector13/13 -> outpmodule/495(VTQD_DriverWhlTqDemFr_Nm)  "<VTQD_DriverWhlTqDemFr_Nm>"
  bus_selector10/2 -> outpmodule/305(VSYS_HWVer2_cnt)  "<VSYS_HWVer2_cnt>"
  BSCP_outputs/1 -> bus_selector9/1
  bus_selector9/27 -> outpmodule/301(VSCP_DTbyte5_raw)  "<VSCP_DTbyte5_raw>"
  outpmodule/590(VOUTP_ACCComfortBandUpper_mps2) -> bus_creator/590
  outpmodule/133(VOUTP_EPBExtReleaseAvail_flg) -> bus_creator/133
  bus_selector13/20 -> outpmodule/502(VTQD_RrEDUSpd_rpm)  "<VTQD_RrEDUSpd_rpm>"
  bus_selector9/26 -> outpmodule/300(VSCP_DTbyte4_raw)  "<VSCP_DTbyte4_raw>"
  bus_selector12/49 -> outpmodule/440(VTPM_S4L_enum)  "<VTPM_S4L_enum>"
  outpmodule/617(VOUTP_ADASLDWMute_flg) -> bus_creator/617
  outpmodule/126(VOUTP_BrkSwStaTimeOut_flg) -> bus_creator/126
  bus_selector9/24 -> outpmodule/298(VSCP_DTbyte2_raw)  "<VSCP_DTbyte2_raw>"
  bus_selector12/83 -> outpmodule/474(VTPM_Flashdatavalid_enum)  "<VTPM_Flashdatavalid_enum>"
  bus_selector9/25 -> outpmodule/299(VSCP_DTbyte3_raw)  "<VSCP_DTbyte3_raw>"
  bus_selector3/31 -> outpmodule/200(VBCM_TgateSWLSta_flg)  "<VBCM_TgateSWLSta_flg>"
  outpmodule/197(VOUTP_RrAtmoLampCmd_flg) -> bus_creator/197
  bus_selector12/59 -> outpmodule/450(VTPM_S3WheelDebugALTU_pct)  "<VTPM_S3WheelDebugALTU_pct>"
  bus_selector13/46 -> outpmodule/528(VTQD_DrvDemEMRtapTrq_pct)  "<VTQD_DrvDemEMRtapTrq_pct>"
  bus_selector12/64 -> outpmodule/455(VTPM_ID4messageALTU_raw8)  "<VTPM_ID4messageALTU_raw8>"
  outpmodule/180(VOUTP_HBeam_flg) -> bus_creator/180
  bus_selector9/22 -> outpmodule/296(VSCP_DTbyte0_raw)  "<VSCP_DTbyte0_raw>"
  bus_selector16/64 -> outpmodule/613(VVMC_ADASLaneModeL_enum)  "<VVMC_ADASLaneModeL_enum>"
  bus_selector3/35 -> outpmodule/204(VBCM_FDDoorOpen_enum)  "<VBCM_FDDoorOpen_enum>"
  outpmodule/330(VOUTP_SHA6_cnt) -> bus_creator/330
  bus_selector10/11 -> outpmodule/314(VSYS_Minor1_cnt)  "<VSYS_Minor1_cnt>"
  outpmodule/335(VOUTP_FdcSlpTime_sec) -> bus_creator/335
  bus_selector2/157 -> outpmodule/164(VAPM_APSHWVer_enum)  "<VAPM_APSHWVer_enum>"
  bus_selector3/30 -> outpmodule/199(VBCM_TgateHDSWRSta_flg)  "<VBCM_TgateHDSWRSta_flg>"
  outpmodule/351(VOUTP_FDAGSCmd_enum) -> bus_creator/351
  bus_selector9/20 -> outpmodule/294(VSCP_CFGEM1BAMPGN_raw)  "<VSCP_CFGEM1BAMPGN_raw>"
  bus_selector9/21 -> outpmodule/295(VSCP_triggerDT_flg)  "<VSCP_triggerDT_flg>"
  outpmodule/124(VOUTP_MCPressureVTimeOut_flg) -> bus_creator/124
  outpmodule/127(VOUTP_BrkSwV_flg) -> bus_creator/127
  bus_selector9/17 -> outpmodule/291(VSCP_CFGEM1BAMTSize_raw)  "<VSCP_CFGEM1BAMTSize_raw>"
  bus_selector3/20 -> outpmodule/189(VBCM_TurnLpRActiveCmd_flg)  "<VBCM_TurnLpRActiveCmd_flg>"
  bus_selector9/19 -> outpmodule/293(VSCP_CFGEM1BAMRsv_raw)  "<VSCP_CFGEM1BAMRsv_raw>"
  outpmodule/301(VOUTP_DTbyte5_raw) -> bus_creator/301
  bus_selector9/16 -> outpmodule/290(VSCP_CFGEM1Ctrl_raw)  "<VSCP_CFGEM1Ctrl_raw>"
  bus_selector13/10 -> outpmodule/492(VTQD_RrActvDmpDisabReq_flg)  "<VTQD_RrActvDmpDisabReq_flg>"
  outpmodule/547(VOUTP_RrTMTqReq_Nm) -> bus_creator/547
  bus_selector9/14 -> outpmodule/288(VSCP_SeatBeltSwitch_enum)  "<VSCP_SeatBeltSwitch_enum>"
  bus_selector12/82 -> outpmodule/473(VTPM_Flashchkdatavalid_enum)  "<VTPM_Flashchkdatavalid_enum>"
  bus_selector9/15 -> outpmodule/289(VSCP_triggerBAM_flg)  "<VSCP_triggerBAM_flg>"
  outpmodule/554(VOUTP_VMCAEBCtrlAvail_flg) -> bus_creator/554
  outpmodule/59(VOUTP_LFRawWhlSpeedV_flg) -> bus_creator/59
  bus_selector13/19 -> outpmodule/501(VTQD_FrEDUSpd_rpm)  "<VTQD_FrEDUSpd_rpm>"
  bus_selector8/47 -> outpmodule/273(VPMM_EHPSRlyDem_enum)  "<VPMM_EHPSRlyDem_enum>"
  bus_selector9/12 -> outpmodule/286(VSCP_OpenStatusOfDoor1_enum)  "<VSCP_OpenStatusOfDoor1_enum>"
  bus_selector8/42 -> outpmodule/268(VPMM_HWResetSta_enum)  "<VPMM_HWResetSta_enum>"
  outpmodule/99(VOUTP_SASSpeed_degps) -> bus_creator/99
  bus_selector13/55 -> outpmodule/537(VTQD_NFricPercTorq_pct)  "<VTQD_NFricPercTorq_pct>"
  bus_selector2/72 -> outpmodule/79(VAPM_LRPulseCountV_flg)  "<VAPM_LRPulseCountV_flg>"
  outpmodule/230(VOUTP_PowerDownFault_enum) -> bus_creator/230
  bus_selector8/46 -> outpmodule/272(VPMM_EACRlyDem_enum)  "<VPMM_EACRlyDem_enum>"
  outpmodule/641(VOUTP_APSDecReqA_flg) -> bus_creator/641
  bus_selector8/45 -> outpmodule/271(VPMM_DCDCRlyDem_enum)  "<VPMM_DCDCRlyDem_enum>"
  outpmodule/489(VOUTP_ShiftGearPosn_enum) -> bus_creator/489
  bus_selector2/24 -> outpmodule/31(VAPM_PASAFML_enum)  "<VAPM_PASAFML_enum>"
  bus_selector8/48 -> outpmodule/274(VPMM_DCDCEnDem_enum)  "<VPMM_DCDCEnDem_enum>"
  bus_selector13/53 -> outpmodule/535(VTQD_VCUVehSpd_kph)  "<VTQD_VCUVehSpd_kph>"
  bus_selector12/40 -> outpmodule/431(VTPM_LRSensorMode_flg)  "<VTPM_LRSensorMode_flg>"
  outpmodule/70(VOUTP_RFWhlRotDirTimeOut_flg) -> bus_creator/70
  bus_selector8/44 -> outpmodule/270(VPMM_PwrStaTOSta_enum)  "<VPMM_PwrStaTOSta_enum>"
  bus_selector8/41 -> outpmodule/267(VPMM_CtrlFrEDUINVERTER_flg)  "<VPMM_CtrlFrEDUINVERTER_flg>"
  outpmodule/56(VOUTP_LRRawWhlSpeedTimeOut_flg) -> bus_creator/56
  bus_selector16/31 -> outpmodule/580(VVMC_ADASAEBReq_enum)  "<VVMC_ADASAEBReq_enum>"
  bus_selector8/40 -> outpmodule/266(VPMM_CtrlFrBMSCCUCIR_flg)  "<VPMM_CtrlFrBMSCCUCIR_flg>"
  bus_selector8/38 -> outpmodule/264(VPMM_CtrlFrPwrStbA1P_flg)  "<VPMM_CtrlFrPwrStbA1P_flg>"
  bus_selector12/10 -> outpmodule/401(VTPM_RFWheelTemp_C)  "<VTPM_RFWheelTemp_C>"
  outpmodule/366(VOUTP_sigAirIntenZon1St_enum) -> bus_creator/366
  bus_selector8/36 -> outpmodule/262(VPMM_LVSilentChrgReq_flg)  "<VPMM_LVSilentChrgReq_flg>"
  bus_selector12/39 -> outpmodule/430(VTPM_RFSensorMode_flg)  "<VTPM_RFSensorMode_flg>"
  bus_selector2/84 -> outpmodule/91(VAPM_ShifterHandleCmd_enum)  "<VAPM_ShifterHandleCmd_enum>"
  bus_selector8/35 -> outpmodule/261(VPMM_LVSilentChrgSta_enum)  "<VPMM_LVSilentChrgSta_enum>"
  outpmodule/12(VOUTP_ChrgPlugSta_enum) -> bus_creator/12
  bus_selector8/34 -> outpmodule/260(VPMM_PMMAllowECUSleep_flg)  "<VPMM_PMMAllowECUSleep_flg>"
  outpmodule/380(VOUTP_Face_flg) -> bus_creator/380
  bus_selector2/147 -> outpmodule/154(VAPM_IVIScreenTimeOut_flg)  "<VAPM_IVIScreenTimeOut_flg>"
  bus_selector16/94 -> outpmodule/643(VVMC_APSReq_enum)  "<VVMC_APSReq_enum>"
  outpmodule/482(VOUTP_FlashIDvalid_enum) -> bus_creator/482
  bus_selector8/39 -> outpmodule/265(VPMM_CtrlFrRC1_flg)  "<VPMM_CtrlFrRC1_flg>"
  bus_selector10/8 -> outpmodule/311(VSYS_ECU2_cnt)  "<VSYS_ECU2_cnt>"
  bus_selector8/9 -> outpmodule/235(VPMM_HVSysReadyToCharge_enum)  "<VPMM_HVSysReadyToCharge_enum>"
  outpmodule/316(VOUTP_Patch1_cnt) -> bus_creator/316
  outpmodule/575(VOUTP_LateralCtrl_flg) -> bus_creator/575
  bus_selector8/37 -> outpmodule/263(VPMM_LVSilentChrgLv_enum)  "<VPMM_LVSilentChrgLv_enum>"
  bus_selector8/27 -> outpmodule/253(VPMM_PwrStaONTOPopReq_flg)  "<VPMM_PwrStaONTOPopReq_flg>"
  outpmodule/119(VOUTP_LatAccelV_flg) -> bus_creator/119
  outpmodule/543(VOUTP_FDCCHAEBSHHSwSta_enum) -> bus_creator/543
  bus_selector13/3 -> outpmodule/485(VTQD_TqSourceRr_enum)  "<VTQD_TqSourceRr_enum>"
  bus_selector8/32 -> outpmodule/258(VPMM_TimerAllowSleep_flg)  "<VPMM_TimerAllowSleep_flg>"
  outpmodule/114(VOUTP_LongAccelTimeOut_flg) -> bus_creator/114
  bus_selector8/31 -> outpmodule/257(VPMM_SilentChkAllowSleep_flg)  "<VPMM_SilentChkAllowSleep_flg>"
  outpmodule/619(VOUTP_ADASLFCHandsOffWarning_enum) -> bus_creator/619
  outpmodule/404(VOUTP_LFSensorFail_flg) -> bus_creator/404
  bus_selector8/33 -> outpmodule/259(VPMM_FDADC12VDetAvg_mV)  "<VPMM_FDADC12VDetAvg_mV>"
  bus_selector12/21 -> outpmodule/412(VTPM_TPMSResButtAllow_flg)  "<VTPM_TPMSResButtAllow_flg>"
  outpmodule/179(VOUTP_RrFogLamp_flg) -> bus_creator/179
  bus_selector8/28 -> outpmodule/254(VPMM_IVIPwrStaONTOPopT_s)  "<VPMM_IVIPwrStaONTOPopT_s>"
  outpmodule/434(VOUTP_S2ID_raw32) -> bus_creator/434
  outpmodule/266(VOUTP_CtrlFrBMSCCUCIR_flg) -> bus_creator/266
  outpmodule/58(VOUTP_RRRawWhlSpeedTimeOut_flg) -> bus_creator/58
  bus_selector2/38 -> outpmodule/45(VAPM_Chime_enum)  "<VAPM_Chime_enum>"
  bus_selector8/25 -> outpmodule/251(VPMM_LVSysErrPwrOutErr_flg)  "<VPMM_LVSysErrPwrOutErr_flg>"
  outpmodule/635(VOUTP_ACCPedalOvrd_flg) -> bus_creator/635
  bus_selector8/26 -> outpmodule/252(VPMM_EvccAplusPwrUpReq_flg)  "<VPMM_EvccAplusPwrUpReq_flg>"
  bus_selector8/18 -> outpmodule/244(VPMM_PwrStaSelect_enum)  "<VPMM_PwrStaSelect_enum>"
  bus_selector10/27 -> outpmodule/330(VSYS_SHA6_cnt)  "<VSYS_SHA6_cnt>"
  outpmodule/427(VOUTP_CWheelTips_enum) -> bus_creator/427
  bus_selector8/19 -> outpmodule/245(VPMM_PwrStaConstraint_enum)  "<VPMM_PwrStaConstraint_enum>"
  bus_selector2/28 -> outpmodule/35(VAPM_USSStaRLR_flg)  "<VAPM_USSStaRLR_flg>"
  bus_selector8/22 -> outpmodule/248(VPMM_PwrDownReq_enum)  "<VPMM_PwrDownReq_enum>"
  bus_selector12/60 -> outpmodule/451(VTPM_S4WheelDebugALTU_pct)  "<VTPM_S4WheelDebugALTU_pct>"
  bus_selector2/8 -> outpmodule/15(VAPM_PASDRCR_cm)  "<VAPM_PASDRCR_cm>"
  bus_selector12/4 -> outpmodule/395(VTPM_RRBatWarn_flg)  "<VTPM_RRBatWarn_flg>"
  bus_selector2/11 -> outpmodule/18(VAPM_PASDFML_cm)  "<VAPM_PASDFML_cm>"
  bus_selector9/13 -> outpmodule/287(VSCP_OpenStatusOfDoor2_enum)  "<VSCP_OpenStatusOfDoor2_enum>"
  bus_selector12/11 -> outpmodule/402(VTPM_LRWheelTemp_C)  "<VTPM_LRWheelTemp_C>"
  outpmodule/54(VOUTP_RFRawWhlSpeedTimeOut_flg) -> bus_creator/54
  outpmodule/625(VOUTP_ADASLFCWarnSound_enum) -> bus_creator/625
  bus_selector2/9 -> outpmodule/16(VAPM_PASDRCL_cm)  "<VAPM_PASDRCL_cm>"
  bus_selector2/145 -> outpmodule/152(VAPM_CAASSwTimeOut_flg)  "<VAPM_CAASSwTimeOut_flg>"
  outpmodule/251(VOUTP_LVSysErrPwrOutErr_flg) -> bus_creator/251
  bus_selector2/6 -> outpmodule/13(VAPM_PASDRMR_cm)  "<VAPM_PASDRMR_cm>"
  bus_selector15/1 -> outpmodule/548(VV2L_ReqOBCV2LEna_enum)  "<VV2L_ReqOBCV2LEna_enum>"
  bus_selector2/7 -> outpmodule/14(VAPM_PASDRML_cm)  "<VAPM_PASDRML_cm>"
  outpmodule/609(VOUTP_ADASSLIFSpdLim_enum) -> bus_creator/609
  bus_selector2/5 -> outpmodule/12(VAPM_ChrgPlugSta_enum)  "<VAPM_ChrgPlugSta_enum>"
  bus_selector8/6 -> outpmodule/232(VPMM_DCDCEnaReq_flg)  "<VPMM_DCDCEnaReq_flg>"
  bus_selector2/33 -> outpmodule/40(VAPM_USSStaFML_flg)  "<VAPM_USSStaFML_flg>"
  outpmodule/620(VOUTP_LVDADisabled_flg) -> bus_creator/620
  outpmodule/156(VOUTP_ABSActiveTimeOut_flg) -> bus_creator/156
  outpmodule/421(VOUTP_LRWheelTmpIndi_flg) -> bus_creator/421
  outpmodule/159(VOUTP_DriverSeatBeltCmd_flg) -> bus_creator/159
  bus_selector16/73 -> outpmodule/622(VVMC_LVDAFailinfo_flg)  "<VVMC_LVDAFailinfo_flg>"
  bus_selector2/10 -> outpmodule/17(VAPM_PASDFMR_cm)  "<VAPM_PASDFMR_cm>"
  bus_selector8/29 -> outpmodule/255(VPMM_LVChrgHoldTtimer_s)  "<VPMM_LVChrgHoldTtimer_s>"
  bus_selector2/158 -> outpmodule/165(VAPM_APSExitCondition_enum)  "<VAPM_APSExitCondition_enum>"
  outpmodule/315(VOUTP_Minor2_cnt) -> bus_creator/315
  bus_selector11/9 -> outpmodule/348(VTHC_FDTWVCmd_pct)  "<VTHC_FDTWVCmd_pct>"
  bus_selector11/8 -> outpmodule/347(VTHC_FDFWVCmd_flg)  "<VTHC_FDFWVCmd_flg>"
  bus_selector11/6 -> outpmodule/345(VTHC_FDEXV2Cmd_step)  "<VTHC_FDEXV2Cmd_step>"
  bus_selector11/5 -> outpmodule/344(VTHC_FDEXV1Cmd_step)  "<VTHC_FDEXV1Cmd_step>"
  outpmodule/598(VOUTP_RightTurnLightReq_flg) -> bus_creator/598
  outpmodule/537(VOUTP_NFricPercTorq_pct) -> bus_creator/537
  bus_selector9/11 -> outpmodule/285(VSCP_BrkPedalPos_pct)  "<VSCP_BrkPedalPos_pct>"
  bus_selector11/4 -> outpmodule/343(VTHC_FDSOV3Cmd_flg)  "<VTHC_FDSOV3Cmd_flg>"
  bus_selector11/3 -> outpmodule/342(VTHC_FDSOV2Cmd_flg)  "<VTHC_FDSOV2Cmd_flg>"
  BVMC_outputs/1 -> bus_selector16/1
  outpmodule/443(VOUTP_RFP20_raw8) -> bus_creator/443
  bus_selector12/13 -> outpmodule/404(VTPM_LFSensorFail_flg)  "<VTPM_LFSensorFail_flg>"
  outpmodule/123(VOUTP_MCPressureV_bar) -> bus_creator/123
  bus_selector11/2 -> outpmodule/341(VTHC_FDSOV1Cmd_flg)  "<VTHC_FDSOV1Cmd_flg>"
  outpmodule/564(VOUTP_SingleWhlSlipRatioCtrl_flg) -> bus_creator/564
  bus_selector13/29 -> outpmodule/511(VTQD_FrIdcMin_A)  "<VTQD_FrIdcMin_A>"
  bus_selector11/1 -> outpmodule/340(VTHC_FDCompCmd_rpm)  "<VTHC_FDCompCmd_rpm>"
  outpmodule/432(VOUTP_RRSensorMode_flg) -> bus_creator/432
  bus_selector8/43 -> outpmodule/269(VPMM_CtrlDrPwrStbA2_flg)  "<VPMM_CtrlDrPwrStbA2_flg>"
  bus_selector2/50 -> outpmodule/57(VAPM_RRRawWhlSpeed_kph)  "<VAPM_RRRawWhlSpeed_kph>"
  bus_selector13/48 -> outpmodule/530(VTQD_RetSelNonEng_pct)  "<VTQD_RetSelNonEng_pct>"
  outpmodule/531(VOUTP_ShiftPgs_enum) -> bus_creator/531
  bus_selector2/117 -> outpmodule/124(VAPM_MCPressureVTimeOut_flg)  "<VAPM_MCPressureVTimeOut_flg>"
  outpmodule/442(VOUTP_LFP20_raw8) -> bus_creator/442
  BSYS_outputs/1 -> bus_selector10/1
  bus_selector9/18 -> outpmodule/292(VSCP_CFGEM1BAMTNum_raw)  "<VSCP_CFGEM1BAMTNum_raw>"
  bus_selector12/48 -> outpmodule/439(VTPM_S3L_enum)  "<VTPM_S3L_enum>"
  bus_selector10/35 -> outpmodule/338(VSYS_AcoreRebootCmdACK_flg)  "<VSYS_AcoreRebootCmdACK_flg>"
  bus_selector2/44 -> outpmodule/51(VAPM_LFRawWhlSpeed_kph)  "<VAPM_LFRawWhlSpeed_kph>"
  outpmodule/498(VOUTP_RrEDUActTq_Nm) -> bus_creator/498
  bus_selector13/22 -> outpmodule/504(VTQD_FrEDUAvailBrkRgnTqV_flg)  "<VTQD_FrEDUAvailBrkRgnTqV_flg>"
  outpmodule/423(VOUTP_LFWheelPSW_raw8) -> bus_creator/423
  bus_selector1/6 -> outpmodule/6(VACC_CACTempWarnSta_flg)  "<VACC_CACTempWarnSta_flg>"
  BPMM_outputs/1 -> bus_selector8/1
  bus_selector10/36 -> outpmodule/339(VSYS_CurrentNmState_enum)  "<VSYS_CurrentNmState_enum>"
  outpmodule/321(VOUTP_Dash1_cnt) -> bus_creator/321
  bus_selector2/130 -> outpmodule/137(VAPM_EPBErrSta_enum)  "<VAPM_EPBErrSta_enum>"
  bus_selector10/34 -> outpmodule/337(VSYS_WisrBootReason_raw32)  "<VSYS_WisrBootReason_raw32>"
  bus_selector16/89 -> outpmodule/638(VVMC_MSACtrlSta_enum)  "<VVMC_MSACtrlSta_enum>"
  bus_selector10/33 -> outpmodule/336(VSYS_PmicBootReason_enum)  "<VSYS_PmicBootReason_enum>"
  bus_selector2/30 -> outpmodule/37(VAPM_USSStaRCR_flg)  "<VAPM_USSStaRCR_flg>"
  bus_selector10/31 -> outpmodule/334(VSYS_FdcSlpReqRisingEdge_flg)  "<VSYS_FdcSlpReqRisingEdge_flg>"
  bus_selector3/13 -> outpmodule/182(VBCM_PosLamp_flg)  "<VBCM_PosLamp_flg>"
  outpmodule/296(VOUTP_DTbyte0_raw) -> bus_creator/296
  outpmodule/370(VOUTP_sigSetTempZon2St_C) -> bus_creator/370
  bus_selector10/32 -> outpmodule/335(VSYS_FdcSlpTime_sec)  "<VSYS_FdcSlpTime_sec>"
  bus_selector11/35 -> outpmodule/374(VTHC_sigCbnSolarRight_W)  "<VTHC_sigCbnSolarRight_W>"
  bus_selector2/36 -> outpmodule/43(VAPM_USSStaFCR_flg)  "<VAPM_USSStaFCR_flg>"
  outpmodule/627(VOUTP_ADASLanetypeR_enum) -> bus_creator/627
  bus_selector11/29 -> outpmodule/368(VTHC_sigRecircSt_flg)  "<VTHC_sigRecircSt_flg>"
  bus_selector8/17 -> outpmodule/243(VPMM_DrSeatSta_enum)  "<VPMM_DrSeatSta_enum>"
  bus_selector16/77 -> outpmodule/626(VVMC_FCMACCmode_enum)  "<VVMC_FCMACCmode_enum>"
  bus_selector11/32 -> outpmodule/371(VTHC_sigClntTHvBattOut_C)  "<VTHC_sigClntTHvBattOut_C>"
  bus_selector12/3 -> outpmodule/394(VTPM_LRBatWarn_flg)  "<VTPM_LRBatWarn_flg>"
  bus_selector2/113 -> outpmodule/120(VAPM_LatAccelVTimeOut_flg)  "<VAPM_LatAccelVTimeOut_flg>"
  bus_selector11/30 -> outpmodule/369(VTHC_sigSetTempZon1St_C)  "<VTHC_sigSetTempZon1St_C>"
  outpmodule/472(VOUTP_WriteChkfinRRID_raw) -> bus_creator/472
  bus_selector3/27 -> outpmodule/196(VBCM_FrAtmoLampCmd_flg)  "<VBCM_FrAtmoLampCmd_flg>"
  outpmodule/406(VOUTP_LRSensorFail_flg) -> bus_creator/406
  bus_selector11/31 -> outpmodule/370(VTHC_sigSetTempZon2St_C)  "<VTHC_sigSetTempZon2St_C>"
  bus_selector8/24 -> outpmodule/250(VPMM_ReVehThdChkSta_enum)  "<VPMM_ReVehThdChkSta_enum>"
  bus_selector11/28 -> outpmodule/367(VTHC_sigWindDirZon1St_enum)  "<VTHC_sigWindDirZon1St_enum>"
  bus_selector13/41 -> outpmodule/523(VTQD_ActDriveDirect_enum)  "<VTQD_ActDriveDirect_enum>"
  bus_selector11/27 -> outpmodule/366(VTHC_sigAirIntenZon1St_enum)  "<VTHC_sigAirIntenZon1St_enum>"
  bus_selector2/54 -> outpmodule/61(VAPM_RFRawWhlSpeedV_flg)  "<VAPM_RFRawWhlSpeedV_flg>"
  bus_selector11/22 -> outpmodule/361(VTHC_CabinMode_enum)  "<VTHC_CabinMode_enum>"
  bus_selector11/21 -> outpmodule/360(VTHC_EDriveMode_enum)  "<VTHC_EDriveMode_enum>"
  bus_selector2/17 -> outpmodule/24(VAPM_APSDFLL_cm)  "<VAPM_APSDFLL_cm>"
  outpmodule/243(VOUTP_DrSeatSta_enum) -> bus_creator/243
  bus_selector11/20 -> outpmodule/359(VTHC_BatteryMode_enum)  "<VTHC_BatteryMode_enum>"
  bus_selector3/6 -> outpmodule/175(VBCM_BrakeLamp_flg)  "<VBCM_BrakeLamp_flg>"
  bus_selector11/17 -> outpmodule/356(VTHC_FDFrRiAPTCHeatPwrCmd_W)  "<VTHC_FDFrRiAPTCHeatPwrCmd_W>"
  bus_selector4/3 -> outpmodule/208(VDHP_EAPS2MIN_pct)  "<VDHP_EAPS2MIN_pct>"
  outpmodule/68(VOUTP_LFWhlRotDirTimeOut_flg) -> bus_creator/68
  outpmodule/514(VOUTP_FrUdcMax_V) -> bus_creator/514
  outpmodule/611(VOUTP_LKAHODSoundWarning_flg) -> bus_creator/611
  outpmodule/203(VOUTP_RTgateRelCmd_flg) -> bus_creator/203
  bus_selector11/18 -> outpmodule/357(VTHC_FDRrAPTCHeatPwrCmd_W)  "<VTHC_FDRrAPTCHeatPwrCmd_W>"
  bus_selector11/16 -> outpmodule/355(VTHC_FDFrLeAPTCHeatPwrCmd_W)  "<VTHC_FDFrLeAPTCHeatPwrCmd_W>"
  outpmodule/90(VOUTP_RRPulseCountTimeOut_flg) -> bus_creator/90
  bus_selector11/13 -> outpmodule/352(VTHC_FDEWP1Cmd_enum)  "<VTHC_FDEWP1Cmd_enum>"
  outpmodule/632(VOUTP_FCMLDWRequest_enum) -> bus_creator/632
  bus_selector2/95 -> outpmodule/102(VAPM_SASSpeedValidTimeOut_flg)  "<VAPM_SASSpeedValidTimeOut_flg>"
  bus_selector11/10 -> outpmodule/349(VTHC_FDFrWPTCHeatPwrCmd_W)  "<VTHC_FDFrWPTCHeatPwrCmd_W>"
  outpmodule/507(VOUTP_RgnAbnorSta_flg) -> bus_creator/507
  bus_selector11/14 -> outpmodule/353(VTHC_FDEWP2Cmd_enum)  "<VTHC_FDEWP2Cmd_enum>"
  outpmodule/475(VOUTP_unlearnSfali_flg) -> bus_creator/475
  bus_selector6/2 -> outpmodule/212(VDSC_DISCTargetSpd_kph)  "<VDSC_DISCTargetSpd_kph>"
  outpmodule/447(VOUTP_IDin_raw32) -> bus_creator/447
  bus_selector11/11 -> outpmodule/350(VTHC_CoolgFanActDuty_pct)  "<VTHC_CoolgFanActDuty_pct>"
  bus_selector6/1 -> outpmodule/211(VDSC_DISCTurn_flg)  "<VDSC_DISCTurn_flg>"
  BDKC_outputs/1 -> bus_selector5/1
  bus_selector7/11 -> outpmodule/225(VNMM_SysNMmSta_enum)  "<VNMM_SysNMmSta_enum>"
  bus_selector13/47 -> outpmodule/529(VTQD_SACtrlDev_enum)  "<VTQD_SACtrlDev_enum>"
  outpmodule/379(VOUTP_ACModeMem_enum) -> bus_creator/379
  bus_selector7/10 -> outpmodule/224(VNMM_ActiveWU_flg)  "<VNMM_ActiveWU_flg>"
  bus_selector11/40 -> outpmodule/379(VTHC_ACModeMem_enum)  "<VTHC_ACModeMem_enum>"
  outpmodule/572(VOUTP_ACCRequiredAccel_mps2) -> bus_creator/572
  bus_selector2/61 -> outpmodule/68(VAPM_LFWhlRotDirTimeOut_flg)  "<VAPM_LFWhlRotDirTimeOut_flg>"
  bus_selector7/8 -> outpmodule/222(VNMM_RptMsgReq_flg)  "<VNMM_RptMsgReq_flg>"
  bus_selector13/4 -> outpmodule/486(VTQD_FrEDUAvailBrkRgnTq_Nm)  "<VTQD_FrEDUAvailBrkRgnTq_Nm>"
  bus_selector7/7 -> outpmodule/221(VNMM_PNI_flg)  "<VNMM_PNI_flg>"
  bus_selector13/58 -> outpmodule/540(VTQD_EEC2MSGCS_raw)  "<VTQD_EEC2MSGCS_raw>"
  outpmodule/569(VOUTP_ISOAccLimit_mps2) -> bus_creator/569
  bus_selector7/4 -> outpmodule/218(VNMM_CSB_flg)  "<VNMM_CSB_flg>"
  bus_selector12/62 -> outpmodule/453(VTPM_ID2messageALTU_raw8)  "<VTPM_ID2messageALTU_raw8>"
  bus_selector9/23 -> outpmodule/297(VSCP_DTbyte1_raw)  "<VSCP_DTbyte1_raw>"
  outpmodule/263(VOUTP_LVSilentChrgLv_enum) -> bus_creator/263
  bus_selector7/2 -> outpmodule/216(VNMM_NMmTxReq_flg)  "<VNMM_NMmTxReq_flg>"
  bus_selector11/24 -> outpmodule/363(VTHC_CCUAutoLampSts_flg)  "<VTHC_CCUAutoLampSts_flg>"
  bus_selector7/3 -> outpmodule/217(VNMM_Awake_enum)  "<VNMM_Awake_enum>"
  outpmodule/398(VOUTP_LRWheelPress_raw8) -> bus_creator/398
  outpmodule/522(VOUTP_ActMaxAvaEMRecpTrq_pct) -> bus_creator/522
  bus_selector16/67 -> outpmodule/616(VVMC_ADASISASta_enum)  "<VVMC_ADASISASta_enum>"
  bus_selector11/19 -> outpmodule/358(VTHC_FDBlowerCmd_pct)  "<VTHC_FDBlowerCmd_pct>"
  bus_selector2/133 -> outpmodule/140(VAPM_EPBStaTimeOut_flg)  "<VAPM_EPBStaTimeOut_flg>"
  bus_selector11/33 -> outpmodule/372(VTHC_sigCbnSolarLeft_W)  "<VTHC_sigCbnSolarLeft_W>"
  bus_selector6/4 -> outpmodule/214(VDSC_DISCButtSta_flg)  "<VDSC_DISCButtSta_flg>"
  outpmodule/525(VOUTP_EMTrqModeDrvBrk_enum) -> bus_creator/525
  bus_selector16/9 -> outpmodule/558(VVMC_FeatArbitrSta_enum)  "<VVMC_FeatArbitrSta_enum>"
  bus_selector12/69 -> outpmodule/460(VTPM_TPMSResButt_flg)  "<VTPM_TPMSResButt_flg>"
  bus_selector11/15 -> outpmodule/354(VTHC_FDEWP3Cmd_enum)  "<VTHC_FDEWP3Cmd_enum>"
  bus_selector9/28 -> outpmodule/302(VSCP_DTbyte6_raw)  "<VSCP_DTbyte6_raw>"
  outpmodule/15(VOUTP_PASDRCR_cm) -> bus_creator/15
  outpmodule/573(VOUTP_DISCReqAcc_mps2) -> bus_creator/573
  bus_selector7/5 -> outpmodule/219(VNMM_ErrorState_enum)  "<VNMM_ErrorState_enum>"
  bus_selector10/7 -> outpmodule/310(VSYS_ECU1_cnt)  "<VSYS_ECU1_cnt>"
  bus_selector9/2 -> outpmodule/276(VSCP_SCPBrkSwSta_flg)  "<VSCP_SCPBrkSwSta_flg>"
  outpmodule/613(VOUTP_ADASLaneModeL_enum) -> bus_creator/613
  outpmodule/223(VOUTP_WakeUp_enum) -> bus_creator/223
  bus_selector2/134 -> outpmodule/141(VAPM_AVMparkingcancel_enum)  "<VAPM_AVMparkingcancel_enum>"
  bus_selector9/1 -> outpmodule/275(VSCP_Vehspeed_kph)  "<VSCP_Vehspeed_kph>"
  BNMM_outputs/1 -> bus_selector7/1
  outpmodule/194(VOUTP_RrRmLampBrightCmd_enum) -> bus_creator/194
  bus_selector9/29 -> outpmodule/303(VSCP_DTbyte7_raw)  "<VSCP_DTbyte7_raw>"
  bus_selector2/162 -> outpmodule/169(VAPM_CAASSta_enum)  "<VAPM_CAASSta_enum>"
  outpmodule/260(VOUTP_PMMAllowECUSleep_flg) -> bus_creator/260
  outpmodule/463(VOUTP_LRPindi_enum) -> bus_creator/463
  bus_selector11/41 -> outpmodule/380(VTHC_Face_flg)  "<VTHC_Face_flg>"
  outpmodule/451(VOUTP_S4WheelDebugALTU_pct) -> bus_creator/451
  bus_selector9/9 -> outpmodule/283(VSCP_HSAActive_flg)  "<VSCP_HSAActive_flg>"
  bus_selector9/10 -> outpmodule/284(VSCP_RedWnlmpSta_flg)  "<VSCP_RedWnlmpSta_flg>"
  BTPM_outputs/1 -> bus_selector12/1
  bus_selector7/1 -> outpmodule/215(VNMM_AllCANTxReq_flg)  "<VNMM_AllCANTxReq_flg>"
  bus_selector6/3 -> outpmodule/213(VDSC_DISCSta_enum)  "<VDSC_DISCSta_enum>"
  outpmodule/503(VOUTP_FrEDUSpdValid_flg) -> bus_creator/503
  bus_selector10/9 -> outpmodule/312(VSYS_Major1_cnt)  "<VSYS_Major1_cnt>"
  bus_selector9/6 -> outpmodule/280(VSCP_MeterIndVehSpeed_kph)  "<VSCP_MeterIndVehSpeed_kph>"
  BDSC_outputs/1 -> bus_selector6/1
  outpmodule/492(VOUTP_RrActvDmpDisabReq_flg) -> bus_creator/492
  outpmodule/14(VOUTP_PASDRML_cm) -> bus_creator/14
  bus_selector10/5 -> outpmodule/308(VSYS_CarModel2_cnt)  "<VSYS_CarModel2_cnt>"
  bus_selector13/1 -> outpmodule/483(VTQD_ParkRequest_flg)  "<VTQD_ParkRequest_flg>"
  bus_selector2/12 -> outpmodule/19(VAPM_PASDFCR_cm)  "<VAPM_PASDFCR_cm>"
  outpmodule/603(VOUTP_ACCObjDstLvl_enum) -> bus_creator/603
  bus_selector9/3 -> outpmodule/277(VSCP_AmberWnlmpSta_flg)  "<VSCP_AmberWnlmpSta_flg>"
  bus_selector3/26 -> outpmodule/195(VBCM_WelcomeDemoSta_flg)  "<VBCM_WelcomeDemoSta_flg>"
  bus_selector9/8 -> outpmodule/282(VSCP_ABSActive_flg)  "<VSCP_ABSActive_flg>"
  outpmodule/546(VOUTP_FrTMTqReq_Nm) -> bus_creator/546
  bus_selector11/23 -> outpmodule/362(VTHC_CCUACLampSts_flg)  "<VTHC_CCUACLampSts_flg>"
  outpmodule/506(VOUTP_RrEDUAvailBrkRgnTqV_flg) -> bus_creator/506
  outpmodule/497(VOUTP_FrEDUActTq_Nm) -> bus_creator/497
  bus_selector10/10 -> outpmodule/313(VSYS_Major2_cnt)  "<VSYS_Major2_cnt>"
  bus_selector12/50 -> outpmodule/441(VTPM_ALFin_flg)  "<VTPM_ALFin_flg>"
  outpmodule/43(VOUTP_USSStaFCR_flg) -> bus_creator/43
  outpmodule/602(VOUTP_ADASFltWrnReq_flg) -> bus_creator/602
  bus_selector16/79 -> outpmodule/628(VVMC_ADASLanetypeL_enum)  "<VVMC_ADASLanetypeL_enum>"
  bus_selector11/26 -> outpmodule/365(VTHC_CCUSyncLampSts_flg)  "<VTHC_CCUSyncLampSts_flg>"
  outpmodule/440(VOUTP_S4L_enum) -> bus_creator/440
  bus_selector16/4 -> outpmodule/553(VVMC_MeterIndSpeed_raw32)  "<VVMC_MeterIndSpeed_raw32>"
  bus_selector9/7 -> outpmodule/281(VSCP_ABSFailed_flg)  "<VSCP_ABSFailed_flg>"
  bus_selector15/2 -> outpmodule/549(VV2L_ReqV2LIVIPopup_enum)  "<VV2L_ReqV2LIVIPopup_enum>"
  outpmodule/615(VOUTP_ADASSLIFSta_enum) -> bus_creator/615
  bus_selector8/23 -> outpmodule/249(VPMM_LowSOCWarn_enum)  "<VPMM_LowSOCWarn_enum>"
  bus_selector13/27 -> outpmodule/509(VTQD_FrRgnPermSta_flg)  "<VTQD_FrRgnPermSta_flg>"
  outpmodule/281(VOUTP_ABSFailed_flg) -> bus_creator/281
  bus_selector9/5 -> outpmodule/279(VSCP_HSAFailed_flg)  "<VSCP_HSAFailed_flg>"
  bus_selector11/25 -> outpmodule/364(VTHC_CCUACMaxLampSts_flg)  "<VTHC_CCUACMaxLampSts_flg>"
  bus_selector2/29 -> outpmodule/36(VAPM_USSStaRLL_flg)  "<VAPM_USSStaRLL_flg>"
  bus_selector8/10 -> outpmodule/236(VPMM_PowerSta_enum)  "<VPMM_PowerSta_enum>"
  outpmodule/17(VOUTP_PASDFMR_cm) -> bus_creator/17
  bus_selector2/32 -> outpmodule/39(VAPM_USSStaFMR_flg)  "<VAPM_USSStaFMR_flg>"
  bus_selector8/30 -> outpmodule/256(VPMM_LVBattChrgTimeCnt_s)  "<VPMM_LVBattChrgTimeCnt_s>"
  outpmodule/450(VOUTP_S3WheelDebugALTU_pct) -> bus_creator/450
  outpmodule/122(VOUTP_LongAccelVTimeOut_flg) -> bus_creator/122
  bus_selector2/3 -> outpmodule/10(VAPM_FSOffSw_enum)  "<VAPM_FSOffSw_enum>"
  bus_selector12/89 -> outpmodule/480(VTPM_FlashS3ID_raw)  "<VTPM_FlashS3ID_raw>"
  outpmodule/273(VOUTP_EHPSRlyDem_enum) -> bus_creator/273
  bus_selector16/58 -> outpmodule/607(VVMC_ADASCAMSpdLim_enum)  "<VVMC_ADASCAMSpdLim_enum>"
  outpmodule/81(VOUTP_RRPulseCountV_flg) -> bus_creator/81
  bus_selector2/1 -> outpmodule/8(VAPM_VehSpeedToAPM_kph)  "<VAPM_VehSpeedToAPM_kph>"
  bus_selector16/66 -> outpmodule/615(VVMC_ADASSLIFSta_enum)  "<VVMC_ADASSLIFSta_enum>"
  bus_selector13/8 -> outpmodule/490(VTQD_PButtonSta_enum)  "<VTQD_PButtonSta_enum>"
  outpmodule/631(VOUTP_ADASAEBSta_enum) -> bus_creator/631
  bus_selector9/4 -> outpmodule/278(VSCP_ABSWnlmpSta_flg)  "<VSCP_ABSWnlmpSta_flg>"
  bus_selector12/47 -> outpmodule/438(VTPM_S2L_enum)  "<VTPM_S2L_enum>"
  bus_selector2/31 -> outpmodule/38(VAPM_USSStaRCL_flg)  "<VAPM_USSStaRCL_flg>"
  bus_selector7/12 -> outpmodule/226(VNMM_NetworkReq_flg)  "<VNMM_NetworkReq_flg>"
  outpmodule/515(VOUTP_RrIdcMin_A) -> bus_creator/515
  bus_selector2/2 -> outpmodule/9(VAPM_VehSpeedTimeOut_flg)  "<VAPM_VehSpeedTimeOut_flg>"
  outpmodule/623(VOUTP_LVDAWarning_flg) -> bus_creator/623
  bus_selector7/9 -> outpmodule/223(VNMM_WakeUp_enum)  "<VNMM_WakeUp_enum>"
  bus_selector13/62 -> outpmodule/544(VTQD_FDCVCUTUpAStaSta_enum)  "<VTQD_FDCVCUTUpAStaSta_enum>"
  bus_selector2/4 -> outpmodule/11(VAPM_FSOffSwTimeOut_flg)  "<VAPM_FSOffSwTimeOut_flg>"
  outpmodule/610(VOUTP_LKAHODDisplayWarning_flg) -> bus_creator/610
  bus_selector2/27 -> outpmodule/34(VAPM_USSStaRML_flg)  "<VAPM_USSStaRML_flg>"
  bus_selector11/7 -> outpmodule/346(VTHC_FDSOTXVCmd_flg)  "<VTHC_FDSOTXVCmd_flg>"
  outpmodule/317(VOUTP_Patch2_cnt) -> bus_creator/317
  outpmodule/118(VOUTP_YawRateVTimeOut_flg) -> bus_creator/118
  bus_selector3/28 -> outpmodule/197(VBCM_RrAtmoLampCmd_flg)  "<VBCM_RrAtmoLampCmd_flg>"
  outpmodule/555(VOUTP_VMCACCCtrlAvail_flg) -> bus_creator/555
  bus_selector11/12 -> outpmodule/351(VTHC_FDAGSCmd_enum)  "<VTHC_FDAGSCmd_enum>"
  bus_selector2/37 -> outpmodule/44(VAPM_USSStaFCL_flg)  "<VAPM_USSStaFCL_flg>"
  outpmodule/253(VOUTP_PwrStaONTOPopReq_flg) -> bus_creator/253
  bus_selector16/62 -> outpmodule/611(VVMC_LKAHODSoundWarning_flg)  "<VVMC_LKAHODSoundWarning_flg>"
  outpmodule/158(VOUTP_TCSActiveTimeOut_flg) -> bus_creator/158
  bus_selector4/1 -> outpmodule/206(VDHP_ActAPSPosn_pct)  "<VDHP_ActAPSPosn_pct>"
  outpmodule/540(VOUTP_EEC2MSGCS_raw) -> bus_creator/540
  bus_selector7/6 -> outpmodule/220(VNMM_NodeID_enum)  "<VNMM_NodeID_enum>"
  outpmodule/339(VOUTP_CurrentNmState_enum) -> bus_creator/339
  bus_selector12/45 -> outpmodule/436(VTPM_S4ID_raw32)  "<VTPM_S4ID_raw32>"
  outpmodule/303(VOUTP_DTbyte7_raw) -> bus_creator/303
  outpmodule/40(VOUTP_USSStaFML_flg) -> bus_creator/40
  bus_selector11/34 -> outpmodule/373(VTHC_sigClntTHvBattIn_C)  "<VTHC_sigClntTHvBattIn_C>"
  bus_selector16/5 -> outpmodule/554(VVMC_VMCAEBCtrlAvail_flg)  "<VVMC_VMCAEBCtrlAvail_flg>"
